simulink model "frbd_64ch_600mhz"  (R2013b)
(part 3 of 148)

  pipeline93 : Subsystem  AncestorBlock=casper_library_delays/pipeline  mask(pipeline){latency=1}
      mask help:
      | An explicitly laid-out delay line to avoid mapping to SRL16s
      | for use in pipelining to help achieve timing closure.
      mask init:
      | pipeline_init(gcb,'latency',latency);
      settings: AttributesFormatString=Latency = %<latency>
      mask Display:
      | port_label('input', 1, 'd');
      | port_label('output', 1, 'q');
      | disp(['Z^-', num2str(latency)]);
  pipeline94 : Subsystem  AncestorBlock=casper_library_delays/pipeline  mask(pipeline){latency=1}
      mask help:
      | An explicitly laid-out delay line to avoid mapping to SRL16s
      | for use in pipelining to help achieve timing closure.
      mask init:
      | pipeline_init(gcb,'latency',latency);
      settings: AttributesFormatString=Latency = %<latency>
      mask Display:
      | port_label('input', 1, 'd');
      | port_label('output', 1, 'q');
      | disp(['Z^-', num2str(latency)]);
  pipeline95 : Subsystem  AncestorBlock=casper_library_delays/pipeline  mask(pipeline){latency=1}
      mask help:
      | An explicitly laid-out delay line to avoid mapping to SRL16s
      | for use in pipelining to help achieve timing closure.
      mask init:
      | pipeline_init(gcb,'latency',latency);
      settings: AttributesFormatString=Latency = %<latency>
      mask Display:
      | port_label('input', 1, 'd');
      | port_label('output', 1, 'q');
      | disp(['Z^-', num2str(latency)]);
  pipeline96 : Subsystem  AncestorBlock=casper_library_delays/pipeline  mask(pipeline){latency=1}
      mask help:
      | An explicitly laid-out delay line to avoid mapping to SRL16s
      | for use in pipelining to help achieve timing closure.
      mask init:
      | pipeline_init(gcb,'latency',latency);
      settings: AttributesFormatString=Latency = %<latency>
      mask Display:
      | port_label('input', 1, 'd');
      | port_label('output', 1, 'q');
      | disp(['Z^-', num2str(latency)]);
  pipeline97 : Subsystem  AncestorBlock=casper_library_delays/pipeline  mask(pipeline){latency=1}
      mask help:
      | An explicitly laid-out delay line to avoid mapping to SRL16s
      | for use in pipelining to help achieve timing closure.
      mask init:
      | pipeline_init(gcb,'latency',latency);
      settings: AttributesFormatString=Latency = %<latency>
      mask Display:
      | port_label('input', 1, 'd');
      | port_label('output', 1, 'q');
      | disp(['Z^-', num2str(latency)]);
  pipeline98 : Subsystem  AncestorBlock=casper_library_delays/pipeline  mask(pipeline){latency=1}
      mask help:
      | An explicitly laid-out delay line to avoid mapping to SRL16s
      | for use in pipelining to help achieve timing closure.
      mask init:
      | pipeline_init(gcb,'latency',latency);
      settings: AttributesFormatString=Latency = %<latency>
      mask Display:
      | port_label('input', 1, 'd');
      | port_label('output', 1, 'q');
      | disp(['Z^-', num2str(latency)]);
  pipeline99 : Subsystem  AncestorBlock=casper_library_delays/pipeline  mask(pipeline){latency=1}
      mask help:
      | An explicitly laid-out delay line to avoid mapping to SRL16s
      | for use in pipelining to help achieve timing closure.
      mask init:
      | pipeline_init(gcb,'latency',latency);
      settings: AttributesFormatString=Latency = %<latency>
      mask Display:
      | port_label('input', 1, 'd');
      | port_label('output', 1, 'q');
      | disp(['Z^-', num2str(latency)]);
  power{1..4} (4 alike) : casper_library_misc/power  BitWidth=18  add_latency=2  mult_latency=3
  ring : Subsystem
  simple_bram_vacc : Subsystem  AncestorBlock=casper_library_accumulators/simple_bram_vacc  mask(simple_bram_vacc){vec_len=16, arith_type=Unsigned, n_bits=26, bin_pt=7}
      mask prompts: vec_len "Vector length:"; arith_type "Output type:"; n_bits "Bit width (output):"; bin_pt "Binary point (output):"
      mask help: This simple vector accumulator is based on a shift register. It outputs its previous accumulated vector after a new_acc pulse is received.
      mask init:
      | simple_bram_vacc_init(gcb, ...
      |     'vec_len', vec_len, ...
      |     'arith_type', arith_type, ...
      |     'n_bits', n_bits, ...
      |     'bin_pt', bin_pt);
      mask TypeOptions arith_type: Signed | Unsigned
  simple_bram_vacc1 : Subsystem  AncestorBlock=casper_library_accumulators/simple_bram_vacc  mask(simple_bram_vacc){vec_len=16, arith_type=Unsigned, n_bits=26, bin_pt=7}
      mask prompts: vec_len "Vector length:"; arith_type "Output type:"; n_bits "Bit width (output):"; bin_pt "Binary point (output):"
      mask help: This simple vector accumulator is based on a shift register. It outputs its previous accumulated vector after a new_acc pulse is received.
      mask init:
      | simple_bram_vacc_init(gcb, ...
      |     'vec_len', vec_len, ...
      |     'arith_type', arith_type, ...
      |     'n_bits', n_bits, ...
      |     'bin_pt', bin_pt);
      mask TypeOptions arith_type: Signed | Unsigned
  simple_bram_vacc10 : Subsystem  AncestorBlock=casper_library_accumulators/simple_bram_vacc  mask(simple_bram_vacc){vec_len=16, arith_type=Unsigned, n_bits=26, bin_pt=7}
      mask prompts: vec_len "Vector length:"; arith_type "Output type:"; n_bits "Bit width (output):"; bin_pt "Binary point (output):"
      mask help: This simple vector accumulator is based on a shift register. It outputs its previous accumulated vector after a new_acc pulse is received.
      mask init:
      | simple_bram_vacc_init(gcb, ...
      |     'vec_len', vec_len, ...
      |     'arith_type', arith_type, ...
      |     'n_bits', n_bits, ...
      |     'bin_pt', bin_pt);
      mask TypeOptions arith_type: Signed | Unsigned
  simple_bram_vacc11 : Subsystem  AncestorBlock=casper_library_accumulators/simple_bram_vacc  mask(simple_bram_vacc){vec_len=16, arith_type=Unsigned, n_bits=26, bin_pt=7}
      mask prompts: vec_len "Vector length:"; arith_type "Output type:"; n_bits "Bit width (output):"; bin_pt "Binary point (output):"
      mask help: This simple vector accumulator is based on a shift register. It outputs its previous accumulated vector after a new_acc pulse is received.
      mask init:
      | simple_bram_vacc_init(gcb, ...
      |     'vec_len', vec_len, ...
      |     'arith_type', arith_type, ...
      |     'n_bits', n_bits, ...
      |     'bin_pt', bin_pt);
      mask TypeOptions arith_type: Signed | Unsigned
  simple_bram_vacc12 : Subsystem  AncestorBlock=casper_library_accumulators/simple_bram_vacc  mask(simple_bram_vacc){vec_len=16, arith_type=Unsigned, n_bits=26, bin_pt=7}
      mask prompts: vec_len "Vector length:"; arith_type "Output type:"; n_bits "Bit width (output):"; bin_pt "Binary point (output):"
      mask help: This simple vector accumulator is based on a shift register. It outputs its previous accumulated vector after a new_acc pulse is received.
      mask init:
      | simple_bram_vacc_init(gcb, ...
      |     'vec_len', vec_len, ...
      |     'arith_type', arith_type, ...
      |     'n_bits', n_bits, ...
      |     'bin_pt', bin_pt);
      mask TypeOptions arith_type: Signed | Unsigned
  simple_bram_vacc13 : Subsystem  AncestorBlock=casper_library_accumulators/simple_bram_vacc  mask(simple_bram_vacc){vec_len=16, arith_type=Unsigned, n_bits=26, bin_pt=7}
      mask prompts: vec_len "Vector length:"; arith_type "Output type:"; n_bits "Bit width (output):"; bin_pt "Binary point (output):"
      mask help: This simple vector accumulator is based on a shift register. It outputs its previous accumulated vector after a new_acc pulse is received.
      mask init:
      | simple_bram_vacc_init(gcb, ...
      |     'vec_len', vec_len, ...
      |     'arith_type', arith_type, ...
      |     'n_bits', n_bits, ...
      |     'bin_pt', bin_pt);
      mask TypeOptions arith_type: Signed | Unsigned
  simple_bram_vacc14 : Subsystem  AncestorBlock=casper_library_accumulators/simple_bram_vacc  mask(simple_bram_vacc){vec_len=16, arith_type=Unsigned, n_bits=26, bin_pt=7}
      mask prompts: vec_len "Vector length:"; arith_type "Output type:"; n_bits "Bit width (output):"; bin_pt "Binary point (output):"
      mask help: This simple vector accumulator is based on a shift register. It outputs its previous accumulated vector after a new_acc pulse is received.
      mask init:
      | simple_bram_vacc_init(gcb, ...
      |     'vec_len', vec_len, ...
      |     'arith_type', arith_type, ...
      |     'n_bits', n_bits, ...
      |     'bin_pt', bin_pt);
      mask TypeOptions arith_type: Signed | Unsigned
  simple_bram_vacc15 : Subsystem  AncestorBlock=casper_library_accumulators/simple_bram_vacc  mask(simple_bram_vacc){vec_len=16, arith_type=Unsigned, n_bits=26, bin_pt=7}
      mask prompts: vec_len "Vector length:"; arith_type "Output type:"; n_bits "Bit width (output):"; bin_pt "Binary point (output):"
      mask help: This simple vector accumulator is based on a shift register. It outputs its previous accumulated vector after a new_acc pulse is received.
      mask init:
      | simple_bram_vacc_init(gcb, ...
      |     'vec_len', vec_len, ...
      |     'arith_type', arith_type, ...
      |     'n_bits', n_bits, ...
      |     'bin_pt', bin_pt);
      mask TypeOptions arith_type: Signed | Unsigned
  simple_bram_vacc16 : Subsystem  AncestorBlock=casper_library_accumulators/simple_bram_vacc  mask(simple_bram_vacc){vec_len=16, arith_type=Unsigned, n_bits=26, bin_pt=7}
      mask prompts: vec_len "Vector length:"; arith_type "Output type:"; n_bits "Bit width (output):"; bin_pt "Binary point (output):"
      mask help: This simple vector accumulator is based on a shift register. It outputs its previous accumulated vector after a new_acc pulse is received.
      mask init:
      | simple_bram_vacc_init(gcb, ...
      |     'vec_len', vec_len, ...
      |     'arith_type', arith_type, ...
      |     'n_bits', n_bits, ...
      |     'bin_pt', bin_pt);
      mask TypeOptions arith_type: Signed | Unsigned
  simple_bram_vacc17 : Subsystem  AncestorBlock=casper_library_accumulators/simple_bram_vacc  mask(simple_bram_vacc){vec_len=16, arith_type=Unsigned, n_bits=26, bin_pt=7}
      mask prompts: vec_len "Vector length:"; arith_type "Output type:"; n_bits "Bit width (output):"; bin_pt "Binary point (output):"
      mask help: This simple vector accumulator is based on a shift register. It outputs its previous accumulated vector after a new_acc pulse is received.
      mask init:
      | simple_bram_vacc_init(gcb, ...
      |     'vec_len', vec_len, ...
      |     'arith_type', arith_type, ...
      |     'n_bits', n_bits, ...
      |     'bin_pt', bin_pt);
      mask TypeOptions arith_type: Signed | Unsigned
  simple_bram_vacc18 : Subsystem  AncestorBlock=casper_library_accumulators/simple_bram_vacc  mask(simple_bram_vacc){vec_len=16, arith_type=Unsigned, n_bits=26, bin_pt=7}
      mask prompts: vec_len "Vector length:"; arith_type "Output type:"; n_bits "Bit width (output):"; bin_pt "Binary point (output):"
      mask help: This simple vector accumulator is based on a shift register. It outputs its previous accumulated vector after a new_acc pulse is received.
      mask init:
      | simple_bram_vacc_init(gcb, ...
      |     'vec_len', vec_len, ...
      |     'arith_type', arith_type, ...
      |     'n_bits', n_bits, ...
      |     'bin_pt', bin_pt);
      mask TypeOptions arith_type: Signed | Unsigned
  simple_bram_vacc19 : Subsystem  AncestorBlock=casper_library_accumulators/simple_bram_vacc  mask(simple_bram_vacc){vec_len=16, arith_type=Unsigned, n_bits=26, bin_pt=7}
      mask prompts: vec_len "Vector length:"; arith_type "Output type:"; n_bits "Bit width (output):"; bin_pt "Binary point (output):"
      mask help: This simple vector accumulator is based on a shift register. It outputs its previous accumulated vector after a new_acc pulse is received.
      mask init:
      | simple_bram_vacc_init(gcb, ...
      |     'vec_len', vec_len, ...
      |     'arith_type', arith_type, ...
      |     'n_bits', n_bits, ...
      |     'bin_pt', bin_pt);
      mask TypeOptions arith_type: Signed | Unsigned
  simple_bram_vacc2 : Subsystem  AncestorBlock=casper_library_accumulators/simple_bram_vacc  mask(simple_bram_vacc){vec_len=16, arith_type=Unsigned, n_bits=26, bin_pt=7}
      mask prompts: vec_len "Vector length:"; arith_type "Output type:"; n_bits "Bit width (output):"; bin_pt "Binary point (output):"
      mask help: This simple vector accumulator is based on a shift register. It outputs its previous accumulated vector after a new_acc pulse is received.
      mask init:
      | simple_bram_vacc_init(gcb, ...
      |     'vec_len', vec_len, ...
      |     'arith_type', arith_type, ...
      |     'n_bits', n_bits, ...
      |     'bin_pt', bin_pt);
      mask TypeOptions arith_type: Signed | Unsigned
  simple_bram_vacc20 : Subsystem  AncestorBlock=casper_library_accumulators/simple_bram_vacc  mask(simple_bram_vacc){vec_len=16, arith_type=Unsigned, n_bits=26, bin_pt=7}
      mask prompts: vec_len "Vector length:"; arith_type "Output type:"; n_bits "Bit width (output):"; bin_pt "Binary point (output):"
      mask help: This simple vector accumulator is based on a shift register. It outputs its previous accumulated vector after a new_acc pulse is received.
      mask init:
      | simple_bram_vacc_init(gcb, ...
      |     'vec_len', vec_len, ...
      |     'arith_type', arith_type, ...
      |     'n_bits', n_bits, ...
      |     'bin_pt', bin_pt);
      mask TypeOptions arith_type: Signed | Unsigned
  simple_bram_vacc21 : Subsystem  AncestorBlock=casper_library_accumulators/simple_bram_vacc  mask(simple_bram_vacc){vec_len=16, arith_type=Unsigned, n_bits=26, bin_pt=7}
      mask prompts: vec_len "Vector length:"; arith_type "Output type:"; n_bits "Bit width (output):"; bin_pt "Binary point (output):"
      mask help: This simple vector accumulator is based on a shift register. It outputs its previous accumulated vector after a new_acc pulse is received.
      mask init:
      | simple_bram_vacc_init(gcb, ...
      |     'vec_len', vec_len, ...
      |     'arith_type', arith_type, ...
      |     'n_bits', n_bits, ...
      |     'bin_pt', bin_pt);
      mask TypeOptions arith_type: Signed | Unsigned
  simple_bram_vacc22 : Subsystem  AncestorBlock=casper_library_accumulators/simple_bram_vacc  mask(simple_bram_vacc){vec_len=16, arith_type=Unsigned, n_bits=26, bin_pt=7}
      mask prompts: vec_len "Vector length:"; arith_type "Output type:"; n_bits "Bit width (output):"; bin_pt "Binary point (output):"
      mask help: This simple vector accumulator is based on a shift register. It outputs its previous accumulated vector after a new_acc pulse is received.
      mask init:
      | simple_bram_vacc_init(gcb, ...
      |     'vec_len', vec_len, ...
      |     'arith_type', arith_type, ...
      |     'n_bits', n_bits, ...
      |     'bin_pt', bin_pt);
      mask TypeOptions arith_type: Signed | Unsigned
  simple_bram_vacc23 : Subsystem  AncestorBlock=casper_library_accumulators/simple_bram_vacc  mask(simple_bram_vacc){vec_len=16, arith_type=Unsigned, n_bits=26, bin_pt=7}
      mask prompts: vec_len "Vector length:"; arith_type "Output type:"; n_bits "Bit width (output):"; bin_pt "Binary point (output):"
      mask help: This simple vector accumulator is based on a shift register. It outputs its previous accumulated vector after a new_acc pulse is received.
      mask init:
      | simple_bram_vacc_init(gcb, ...
      |     'vec_len', vec_len, ...
      |     'arith_type', arith_type, ...
      |     'n_bits', n_bits, ...
      |     'bin_pt', bin_pt);
      mask TypeOptions arith_type: Signed | Unsigned
  simple_bram_vacc24 : Subsystem  AncestorBlock=casper_library_accumulators/simple_bram_vacc  mask(simple_bram_vacc){vec_len=16, arith_type=Unsigned, n_bits=26, bin_pt=7}
      mask prompts: vec_len "Vector length:"; arith_type "Output type:"; n_bits "Bit width (output):"; bin_pt "Binary point (output):"
      mask help: This simple vector accumulator is based on a shift register. It outputs its previous accumulated vector after a new_acc pulse is received.
      mask init:
      | simple_bram_vacc_init(gcb, ...
      |     'vec_len', vec_len, ...
      |     'arith_type', arith_type, ...
      |     'n_bits', n_bits, ...
      |     'bin_pt', bin_pt);
      mask TypeOptions arith_type: Signed | Unsigned
  simple_bram_vacc25 : Subsystem  AncestorBlock=casper_library_accumulators/simple_bram_vacc  mask(simple_bram_vacc){vec_len=16, arith_type=Unsigned, n_bits=26, bin_pt=7}
      mask prompts: vec_len "Vector length:"; arith_type "Output type:"; n_bits "Bit width (output):"; bin_pt "Binary point (output):"
      mask help: This simple vector accumulator is based on a shift register. It outputs its previous accumulated vector after a new_acc pulse is received.
      mask init:
      | simple_bram_vacc_init(gcb, ...
      |     'vec_len', vec_len, ...
      |     'arith_type', arith_type, ...
      |     'n_bits', n_bits, ...
      |     'bin_pt', bin_pt);
      mask TypeOptions arith_type: Signed | Unsigned
  simple_bram_vacc26 : Subsystem  AncestorBlock=casper_library_accumulators/simple_bram_vacc  mask(simple_bram_vacc){vec_len=16, arith_type=Unsigned, n_bits=26, bin_pt=7}
      mask prompts: vec_len "Vector length:"; arith_type "Output type:"; n_bits "Bit width (output):"; bin_pt "Binary point (output):"
      mask help: This simple vector accumulator is based on a shift register. It outputs its previous accumulated vector after a new_acc pulse is received.
      mask init:
      | simple_bram_vacc_init(gcb, ...
      |     'vec_len', vec_len, ...
      |     'arith_type', arith_type, ...
      |     'n_bits', n_bits, ...
      |     'bin_pt', bin_pt);
      mask TypeOptions arith_type: Signed | Unsigned
  simple_bram_vacc27 : Subsystem  AncestorBlock=casper_library_accumulators/simple_bram_vacc  mask(simple_bram_vacc){vec_len=16, arith_type=Unsigned, n_bits=26, bin_pt=7}
      mask prompts: vec_len "Vector length:"; arith_type "Output type:"; n_bits "Bit width (output):"; bin_pt "Binary point (output):"
      mask help: This simple vector accumulator is based on a shift register. It outputs its previous accumulated vector after a new_acc pulse is received.
      mask init:
      | simple_bram_vacc_init(gcb, ...
      |     'vec_len', vec_len, ...
      |     'arith_type', arith_type, ...
      |     'n_bits', n_bits, ...
      |     'bin_pt', bin_pt);
      mask TypeOptions arith_type: Signed | Unsigned
  simple_bram_vacc28 : Subsystem  AncestorBlock=casper_library_accumulators/simple_bram_vacc  mask(simple_bram_vacc){vec_len=16, arith_type=Unsigned, n_bits=26, bin_pt=7}
      mask prompts: vec_len "Vector length:"; arith_type "Output type:"; n_bits "Bit width (output):"; bin_pt "Binary point (output):"
      mask help: This simple vector accumulator is based on a shift register. It outputs its previous accumulated vector after a new_acc pulse is received.
      mask init:
      | simple_bram_vacc_init(gcb, ...
      |     'vec_len', vec_len, ...
      |     'arith_type', arith_type, ...
      |     'n_bits', n_bits, ...
      |     'bin_pt', bin_pt);
      mask TypeOptions arith_type: Signed | Unsigned
  simple_bram_vacc29 : Subsystem  AncestorBlock=casper_library_accumulators/simple_bram_vacc  mask(simple_bram_vacc){vec_len=16, arith_type=Unsigned, n_bits=26, bin_pt=7}
      mask prompts: vec_len "Vector length:"; arith_type "Output type:"; n_bits "Bit width (output):"; bin_pt "Binary point (output):"
      mask help: This simple vector accumulator is based on a shift register. It outputs its previous accumulated vector after a new_acc pulse is received.
      mask init:
      | simple_bram_vacc_init(gcb, ...
      |     'vec_len', vec_len, ...
      |     'arith_type', arith_type, ...
      |     'n_bits', n_bits, ...
      |     'bin_pt', bin_pt);
      mask TypeOptions arith_type: Signed | Unsigned
  simple_bram_vacc3 : Subsystem  AncestorBlock=casper_library_accumulators/simple_bram_vacc  mask(simple_bram_vacc){vec_len=16, arith_type=Unsigned, n_bits=26, bin_pt=7}
      mask prompts: vec_len "Vector length:"; arith_type "Output type:"; n_bits "Bit width (output):"; bin_pt "Binary point (output):"
      mask help: This simple vector accumulator is based on a shift register. It outputs its previous accumulated vector after a new_acc pulse is received.
      mask init:
      | simple_bram_vacc_init(gcb, ...
      |     'vec_len', vec_len, ...
      |     'arith_type', arith_type, ...
      |     'n_bits', n_bits, ...
      |     'bin_pt', bin_pt);
      mask TypeOptions arith_type: Signed | Unsigned
  simple_bram_vacc30 : Subsystem  AncestorBlock=casper_library_accumulators/simple_bram_vacc  mask(simple_bram_vacc){vec_len=16, arith_type=Unsigned, n_bits=26, bin_pt=7}
      mask prompts: vec_len "Vector length:"; arith_type "Output type:"; n_bits "Bit width (output):"; bin_pt "Binary point (output):"
      mask help: This simple vector accumulator is based on a shift register. It outputs its previous accumulated vector after a new_acc pulse is received.
      mask init:
      | simple_bram_vacc_init(gcb, ...
      |     'vec_len', vec_len, ...
      |     'arith_type', arith_type, ...
      |     'n_bits', n_bits, ...
      |     'bin_pt', bin_pt);
      mask TypeOptions arith_type: Signed | Unsigned
  simple_bram_vacc31 : Subsystem  AncestorBlock=casper_library_accumulators/simple_bram_vacc  mask(simple_bram_vacc){vec_len=16, arith_type=Unsigned, n_bits=26, bin_pt=7}
      mask prompts: vec_len "Vector length:"; arith_type "Output type:"; n_bits "Bit width (output):"; bin_pt "Binary point (output):"
      mask help: This simple vector accumulator is based on a shift register. It outputs its previous accumulated vector after a new_acc pulse is received.
      mask init:
      | simple_bram_vacc_init(gcb, ...
      |     'vec_len', vec_len, ...
      |     'arith_type', arith_type, ...
      |     'n_bits', n_bits, ...
      |     'bin_pt', bin_pt);
      mask TypeOptions arith_type: Signed | Unsigned
  simple_bram_vacc32 : Subsystem  AncestorBlock=casper_library_accumulators/simple_bram_vacc  mask(simple_bram_vacc){vec_len=16, arith_type=Unsigned, n_bits=26, bin_pt=7}
      mask prompts: vec_len "Vector length:"; arith_type "Output type:"; n_bits "Bit width (output):"; bin_pt "Binary point (output):"
      mask help: This simple vector accumulator is based on a shift register. It outputs its previous accumulated vector after a new_acc pulse is received.
      mask init:
      | simple_bram_vacc_init(gcb, ...
      |     'vec_len', vec_len, ...
      |     'arith_type', arith_type, ...
      |     'n_bits', n_bits, ...
      |     'bin_pt', bin_pt);
      mask TypeOptions arith_type: Signed | Unsigned
  simple_bram_vacc33 : Subsystem  AncestorBlock=casper_library_accumulators/simple_bram_vacc  mask(simple_bram_vacc){vec_len=16, arith_type=Unsigned, n_bits=26, bin_pt=7}
      mask prompts: vec_len "Vector length:"; arith_type "Output type:"; n_bits "Bit width (output):"; bin_pt "Binary point (output):"
      mask help: This simple vector accumulator is based on a shift register. It outputs its previous accumulated vector after a new_acc pulse is received.
      mask init:
      | simple_bram_vacc_init(gcb, ...
      |     'vec_len', vec_len, ...
      |     'arith_type', arith_type, ...
      |     'n_bits', n_bits, ...
      |     'bin_pt', bin_pt);
      mask TypeOptions arith_type: Signed | Unsigned
  simple_bram_vacc34 : Subsystem  AncestorBlock=casper_library_accumulators/simple_bram_vacc  mask(simple_bram_vacc){vec_len=16, arith_type=Unsigned, n_bits=26, bin_pt=7}
      mask prompts: vec_len "Vector length:"; arith_type "Output type:"; n_bits "Bit width (output):"; bin_pt "Binary point (output):"
      mask help: This simple vector accumulator is based on a shift register. It outputs its previous accumulated vector after a new_acc pulse is received.
      mask init:
      | simple_bram_vacc_init(gcb, ...
      |     'vec_len', vec_len, ...
      |     'arith_type', arith_type, ...
      |     'n_bits', n_bits, ...
      |     'bin_pt', bin_pt);
      mask TypeOptions arith_type: Signed | Unsigned
  simple_bram_vacc35 : Subsystem  AncestorBlock=casper_library_accumulators/simple_bram_vacc  mask(simple_bram_vacc){vec_len=16, arith_type=Unsigned, n_bits=26, bin_pt=7}
      mask prompts: vec_len "Vector length:"; arith_type "Output type:"; n_bits "Bit width (output):"; bin_pt "Binary point (output):"
      mask help: This simple vector accumulator is based on a shift register. It outputs its previous accumulated vector after a new_acc pulse is received.
      mask init:
      | simple_bram_vacc_init(gcb, ...
      |     'vec_len', vec_len, ...
      |     'arith_type', arith_type, ...
      |     'n_bits', n_bits, ...
      |     'bin_pt', bin_pt);
      mask TypeOptions arith_type: Signed | Unsigned
  simple_bram_vacc36 : Subsystem  AncestorBlock=casper_library_accumulators/simple_bram_vacc  mask(simple_bram_vacc){vec_len=16, arith_type=Unsigned, n_bits=26, bin_pt=7}
      mask prompts: vec_len "Vector length:"; arith_type "Output type:"; n_bits "Bit width (output):"; bin_pt "Binary point (output):"
      mask help: This simple vector accumulator is based on a shift register. It outputs its previous accumulated vector after a new_acc pulse is received.
      mask init:
      | simple_bram_vacc_init(gcb, ...
      |     'vec_len', vec_len, ...
      |     'arith_type', arith_type, ...
      |     'n_bits', n_bits, ...
      |     'bin_pt', bin_pt);
      mask TypeOptions arith_type: Signed | Unsigned
  simple_bram_vacc37 : Subsystem  AncestorBlock=casper_library_accumulators/simple_bram_vacc  mask(simple_bram_vacc){vec_len=16, arith_type=Unsigned, n_bits=26, bin_pt=7}
      mask prompts: vec_len "Vector length:"; arith_type "Output type:"; n_bits "Bit width (output):"; bin_pt "Binary point (output):"
      mask help: This simple vector accumulator is based on a shift register. It outputs its previous accumulated vector after a new_acc pulse is received.
      mask init:
      | simple_bram_vacc_init(gcb, ...
      |     'vec_len', vec_len, ...
      |     'arith_type', arith_type, ...
      |     'n_bits', n_bits, ...
      |     'bin_pt', bin_pt);
      mask TypeOptions arith_type: Signed | Unsigned
  simple_bram_vacc38 : Subsystem  AncestorBlock=casper_library_accumulators/simple_bram_vacc  mask(simple_bram_vacc){vec_len=16, arith_type=Unsigned, n_bits=26, bin_pt=7}
      mask prompts: vec_len "Vector length:"; arith_type "Output type:"; n_bits "Bit width (output):"; bin_pt "Binary point (output):"
      mask help: This simple vector accumulator is based on a shift register. It outputs its previous accumulated vector after a new_acc pulse is received.
      mask init:
      | simple_bram_vacc_init(gcb, ...
      |     'vec_len', vec_len, ...
      |     'arith_type', arith_type, ...
      |     'n_bits', n_bits, ...
      |     'bin_pt', bin_pt);
      mask TypeOptions arith_type: Signed | Unsigned
  simple_bram_vacc39 : Subsystem  AncestorBlock=casper_library_accumulators/simple_bram_vacc  mask(simple_bram_vacc){vec_len=16, arith_type=Unsigned, n_bits=26, bin_pt=7}
      mask prompts: vec_len "Vector length:"; arith_type "Output type:"; n_bits "Bit width (output):"; bin_pt "Binary point (output):"
      mask help: This simple vector accumulator is based on a shift register. It outputs its previous accumulated vector after a new_acc pulse is received.
      mask init:
      | simple_bram_vacc_init(gcb, ...
      |     'vec_len', vec_len, ...
      |     'arith_type', arith_type, ...
      |     'n_bits', n_bits, ...
      |     'bin_pt', bin_pt);
      mask TypeOptions arith_type: Signed | Unsigned
  simple_bram_vacc4 : Subsystem  AncestorBlock=casper_library_accumulators/simple_bram_vacc  mask(simple_bram_vacc){vec_len=16, arith_type=Unsigned, n_bits=26, bin_pt=7}
      mask prompts: vec_len "Vector length:"; arith_type "Output type:"; n_bits "Bit width (output):"; bin_pt "Binary point (output):"
      mask help: This simple vector accumulator is based on a shift register. It outputs its previous accumulated vector after a new_acc pulse is received.
      mask init:
      | simple_bram_vacc_init(gcb, ...
      |     'vec_len', vec_len, ...
      |     'arith_type', arith_type, ...
      |     'n_bits', n_bits, ...
      |     'bin_pt', bin_pt);
      mask TypeOptions arith_type: Signed | Unsigned
  simple_bram_vacc40 : Subsystem  AncestorBlock=casper_library_accumulators/simple_bram_vacc  mask(simple_bram_vacc){vec_len=16, arith_type=Unsigned, n_bits=26, bin_pt=7}
      mask prompts: vec_len "Vector length:"; arith_type "Output type:"; n_bits "Bit width (output):"; bin_pt "Binary point (output):"
      mask help: This simple vector accumulator is based on a shift register. It outputs its previous accumulated vector after a new_acc pulse is received.
      mask init:
      | simple_bram_vacc_init(gcb, ...
      |     'vec_len', vec_len, ...
      |     'arith_type', arith_type, ...
      |     'n_bits', n_bits, ...
      |     'bin_pt', bin_pt);
      mask TypeOptions arith_type: Signed | Unsigned
  simple_bram_vacc41 : Subsystem  AncestorBlock=casper_library_accumulators/simple_bram_vacc  mask(simple_bram_vacc){vec_len=16, arith_type=Unsigned, n_bits=26, bin_pt=7}
      mask prompts: vec_len "Vector length:"; arith_type "Output type:"; n_bits "Bit width (output):"; bin_pt "Binary point (output):"
      mask help: This simple vector accumulator is based on a shift register. It outputs its previous accumulated vector after a new_acc pulse is received.
      mask init:
      | simple_bram_vacc_init(gcb, ...
      |     'vec_len', vec_len, ...
      |     'arith_type', arith_type, ...
      |     'n_bits', n_bits, ...
      |     'bin_pt', bin_pt);
      mask TypeOptions arith_type: Signed | Unsigned
  simple_bram_vacc42 : Subsystem  AncestorBlock=casper_library_accumulators/simple_bram_vacc  mask(simple_bram_vacc){vec_len=16, arith_type=Unsigned, n_bits=26, bin_pt=7}
      mask prompts: vec_len "Vector length:"; arith_type "Output type:"; n_bits "Bit width (output):"; bin_pt "Binary point (output):"
      mask help: This simple vector accumulator is based on a shift register. It outputs its previous accumulated vector after a new_acc pulse is received.
      mask init:
      | simple_bram_vacc_init(gcb, ...
      |     'vec_len', vec_len, ...
      |     'arith_type', arith_type, ...
      |     'n_bits', n_bits, ...
      |     'bin_pt', bin_pt);
      mask TypeOptions arith_type: Signed | Unsigned
  simple_bram_vacc43 : Subsystem  AncestorBlock=casper_library_accumulators/simple_bram_vacc  mask(simple_bram_vacc){vec_len=16, arith_type=Unsigned, n_bits=64, bin_pt=35}
      mask prompts: vec_len "Vector length:"; arith_type "Output type:"; n_bits "Bit width (output):"; bin_pt "Binary point (output):"
      mask help: This simple vector accumulator is based on a shift register. It outputs its previous accumulated vector after a new_acc pulse is received.
      mask init:
      | simple_bram_vacc_init(gcb, ...
      |     'vec_len', vec_len, ...
      |     'arith_type', arith_type, ...
      |     'n_bits', n_bits, ...
      |     'bin_pt', bin_pt);
      mask TypeOptions arith_type: Signed | Unsigned
  simple_bram_vacc44 : Subsystem  AncestorBlock=casper_library_accumulators/simple_bram_vacc  mask(simple_bram_vacc){vec_len=16, arith_type=Unsigned, n_bits=64, bin_pt=35}
      mask prompts: vec_len "Vector length:"; arith_type "Output type:"; n_bits "Bit width (output):"; bin_pt "Binary point (output):"
      mask help: This simple vector accumulator is based on a shift register. It outputs its previous accumulated vector after a new_acc pulse is received.
      mask init:
      | simple_bram_vacc_init(gcb, ...
      |     'vec_len', vec_len, ...
      |     'arith_type', arith_type, ...
      |     'n_bits', n_bits, ...
      |     'bin_pt', bin_pt);
      mask TypeOptions arith_type: Signed | Unsigned
  simple_bram_vacc45 : Subsystem  AncestorBlock=casper_library_accumulators/simple_bram_vacc  mask(simple_bram_vacc){vec_len=16, arith_type=Unsigned, n_bits=64, bin_pt=35}
      mask prompts: vec_len "Vector length:"; arith_type "Output type:"; n_bits "Bit width (output):"; bin_pt "Binary point (output):"
      mask help: This simple vector accumulator is based on a shift register. It outputs its previous accumulated vector after a new_acc pulse is received.
      mask init:
      | simple_bram_vacc_init(gcb, ...
      |     'vec_len', vec_len, ...
      |     'arith_type', arith_type, ...
      |     'n_bits', n_bits, ...
      |     'bin_pt', bin_pt);
      mask TypeOptions arith_type: Signed | Unsigned
  simple_bram_vacc46 : Subsystem  AncestorBlock=casper_library_accumulators/simple_bram_vacc  mask(simple_bram_vacc){vec_len=16, arith_type=Unsigned, n_bits=64, bin_pt=35}
      mask prompts: vec_len "Vector length:"; arith_type "Output type:"; n_bits "Bit width (output):"; bin_pt "Binary point (output):"
      mask help: This simple vector accumulator is based on a shift register. It outputs its previous accumulated vector after a new_acc pulse is received.
      mask init:
      | simple_bram_vacc_init(gcb, ...
      |     'vec_len', vec_len, ...
      |     'arith_type', arith_type, ...
      |     'n_bits', n_bits, ...
      |     'bin_pt', bin_pt);
      mask TypeOptions arith_type: Signed | Unsigned
  simple_bram_vacc47 : Subsystem  AncestorBlock=casper_library_accumulators/simple_bram_vacc  mask(simple_bram_vacc){vec_len=16, arith_type=Unsigned, n_bits=26, bin_pt=7}
      mask prompts: vec_len "Vector length:"; arith_type "Output type:"; n_bits "Bit width (output):"; bin_pt "Binary point (output):"
      mask help: This simple vector accumulator is based on a shift register. It outputs its previous accumulated vector after a new_acc pulse is received.
      mask init:
      | simple_bram_vacc_init(gcb, ...
      |     'vec_len', vec_len, ...
      |     'arith_type', arith_type, ...
      |     'n_bits', n_bits, ...
      |     'bin_pt', bin_pt);
      mask TypeOptions arith_type: Signed | Unsigned
  simple_bram_vacc48 : Subsystem  AncestorBlock=casper_library_accumulators/simple_bram_vacc  mask(simple_bram_vacc){vec_len=16, arith_type=Unsigned, n_bits=26, bin_pt=7}
      mask prompts: vec_len "Vector length:"; arith_type "Output type:"; n_bits "Bit width (output):"; bin_pt "Binary point (output):"
      mask help: This simple vector accumulator is based on a shift register. It outputs its previous accumulated vector after a new_acc pulse is received.
      mask init:
      | simple_bram_vacc_init(gcb, ...
      |     'vec_len', vec_len, ...
      |     'arith_type', arith_type, ...
      |     'n_bits', n_bits, ...
      |     'bin_pt', bin_pt);
      mask TypeOptions arith_type: Signed | Unsigned
  simple_bram_vacc49 : Subsystem  AncestorBlock=casper_library_accumulators/simple_bram_vacc  mask(simple_bram_vacc){vec_len=16, arith_type=Unsigned, n_bits=26, bin_pt=7}
      mask prompts: vec_len "Vector length:"; arith_type "Output type:"; n_bits "Bit width (output):"; bin_pt "Binary point (output):"
      mask help: This simple vector accumulator is based on a shift register. It outputs its previous accumulated vector after a new_acc pulse is received.
      mask init:
      | simple_bram_vacc_init(gcb, ...
      |     'vec_len', vec_len, ...
      |     'arith_type', arith_type, ...
      |     'n_bits', n_bits, ...
      |     'bin_pt', bin_pt);
      mask TypeOptions arith_type: Signed | Unsigned
  simple_bram_vacc5 : Subsystem  AncestorBlock=casper_library_accumulators/simple_bram_vacc  mask(simple_bram_vacc){vec_len=16, arith_type=Unsigned, n_bits=26, bin_pt=7}
      mask prompts: vec_len "Vector length:"; arith_type "Output type:"; n_bits "Bit width (output):"; bin_pt "Binary point (output):"
      mask help: This simple vector accumulator is based on a shift register. It outputs its previous accumulated vector after a new_acc pulse is received.
      mask init:
      | simple_bram_vacc_init(gcb, ...
      |     'vec_len', vec_len, ...
      |     'arith_type', arith_type, ...
      |     'n_bits', n_bits, ...
      |     'bin_pt', bin_pt);
      mask TypeOptions arith_type: Signed | Unsigned
  simple_bram_vacc50 : Subsystem  AncestorBlock=casper_library_accumulators/simple_bram_vacc  mask(simple_bram_vacc){vec_len=16, arith_type=Unsigned, n_bits=26, bin_pt=7}
      mask prompts: vec_len "Vector length:"; arith_type "Output type:"; n_bits "Bit width (output):"; bin_pt "Binary point (output):"
      mask help: This simple vector accumulator is based on a shift register. It outputs its previous accumulated vector after a new_acc pulse is received.
      mask init:
      | simple_bram_vacc_init(gcb, ...
      |     'vec_len', vec_len, ...
      |     'arith_type', arith_type, ...
      |     'n_bits', n_bits, ...
      |     'bin_pt', bin_pt);
      mask TypeOptions arith_type: Signed | Unsigned
  simple_bram_vacc6 : Subsystem  AncestorBlock=casper_library_accumulators/simple_bram_vacc  mask(simple_bram_vacc){vec_len=16, arith_type=Unsigned, n_bits=26, bin_pt=7}
      mask prompts: vec_len "Vector length:"; arith_type "Output type:"; n_bits "Bit width (output):"; bin_pt "Binary point (output):"
      mask help: This simple vector accumulator is based on a shift register. It outputs its previous accumulated vector after a new_acc pulse is received.
      mask init:
      | simple_bram_vacc_init(gcb, ...
      |     'vec_len', vec_len, ...
      |     'arith_type', arith_type, ...
      |     'n_bits', n_bits, ...
      |     'bin_pt', bin_pt);
      mask TypeOptions arith_type: Signed | Unsigned
  simple_bram_vacc7 : Subsystem  AncestorBlock=casper_library_accumulators/simple_bram_vacc  mask(simple_bram_vacc){vec_len=16, arith_type=Unsigned, n_bits=26, bin_pt=7}
      mask prompts: vec_len "Vector length:"; arith_type "Output type:"; n_bits "Bit width (output):"; bin_pt "Binary point (output):"
      mask help: This simple vector accumulator is based on a shift register. It outputs its previous accumulated vector after a new_acc pulse is received.
      mask init:
      | simple_bram_vacc_init(gcb, ...
      |     'vec_len', vec_len, ...
      |     'arith_type', arith_type, ...
      |     'n_bits', n_bits, ...
      |     'bin_pt', bin_pt);
      mask TypeOptions arith_type: Signed | Unsigned
  simple_bram_vacc8 : Subsystem  AncestorBlock=casper_library_accumulators/simple_bram_vacc  mask(simple_bram_vacc){vec_len=16, arith_type=Unsigned, n_bits=26, bin_pt=7}
      mask prompts: vec_len "Vector length:"; arith_type "Output type:"; n_bits "Bit width (output):"; bin_pt "Binary point (output):"
      mask help: This simple vector accumulator is based on a shift register. It outputs its previous accumulated vector after a new_acc pulse is received.
      mask init:
      | simple_bram_vacc_init(gcb, ...
      |     'vec_len', vec_len, ...
      |     'arith_type', arith_type, ...
      |     'n_bits', n_bits, ...
      |     'bin_pt', bin_pt);
      mask TypeOptions arith_type: Signed | Unsigned
  simple_bram_vacc86 : Subsystem  AncestorBlock=casper_library_accumulators/simple_bram_vacc  mask(simple_bram_vacc){vec_len=16, arith_type=Unsigned, n_bits=26, bin_pt=7}
      mask prompts: vec_len "Vector length:"; arith_type "Output type:"; n_bits "Bit width (output):"; bin_pt "Binary point (output):"
      mask help: This simple vector accumulator is based on a shift register. It outputs its previous accumulated vector after a new_acc pulse is received.
      mask init:
      | simple_bram_vacc_init(gcb, ...
      |     'vec_len', vec_len, ...
      |     'arith_type', arith_type, ...
      |     'n_bits', n_bits, ...
      |     'bin_pt', bin_pt);
      mask TypeOptions arith_type: Signed | Unsigned
  simple_bram_vacc9 : Subsystem  AncestorBlock=casper_library_accumulators/simple_bram_vacc  mask(simple_bram_vacc){vec_len=16, arith_type=Unsigned, n_bits=26, bin_pt=7}
      mask prompts: vec_len "Vector length:"; arith_type "Output type:"; n_bits "Bit width (output):"; bin_pt "Binary point (output):"
      mask help: This simple vector accumulator is based on a shift register. It outputs its previous accumulated vector after a new_acc pulse is received.
      mask init:
      | simple_bram_vacc_init(gcb, ...
      |     'vec_len', vec_len, ...
      |     'arith_type', arith_type, ...
      |     'n_bits', n_bits, ...
      |     'bin_pt', bin_pt);
      mask TypeOptions arith_type: Signed | Unsigned
  spec0_0 : Subsystem  Tag=xps:bram  AncestorBlock=xps_library/Shared_BRAM  mask{arith_type=Unsigned, addr_width=10, data_width=32, reg_prim_output=on, reg_core_output=on, optimization=Minimum_Area, data_bin_pt=0, init_vals=[0:2^10-1], sample_rate=1}
      mask prompts: arith_type "Output Data Type"; addr_width "Address width"; data_width "Data Width"; reg_prim_output "Register Primitive Output"; reg_core_output "Register Core Output"; data_bin_pt "Data Binary Point"; init_vals "Initial values (simulation only)"; sample_rate "Sample rate"
      mask init:
      | shared_bram_mask;
      mask TypeOptions arith_type: Unsigned | Signed  (2's comp)
      mask TypeOptions data_width: 8 | 16 | 32 | 64 | 128
      mask TypeOptions optimization: Minimum_Area | Low_Power
  spec0_1 : Subsystem  Tag=xps:bram  AncestorBlock=xps_library/Shared_BRAM  mask{arith_type=Unsigned, addr_width=10, data_width=32, reg_prim_output=on, reg_core_output=on, optimization=Minimum_Area, data_bin_pt=0, init_vals=[0:2^10-1], sample_rate=1}
      mask prompts: arith_type "Output Data Type"; addr_width "Address width"; data_width "Data Width"; reg_prim_output "Register Primitive Output"; reg_core_output "Register Core Output"; data_bin_pt "Data Binary Point"; init_vals "Initial values (simulation only)"; sample_rate "Sample rate"
      mask init:
      | shared_bram_mask;
      mask TypeOptions arith_type: Unsigned | Signed  (2's comp)
      mask TypeOptions data_width: 8 | 16 | 32 | 64 | 128
      mask TypeOptions optimization: Minimum_Area | Low_Power
  spec0_2 : Subsystem  Tag=xps:bram  AncestorBlock=xps_library/Shared_BRAM  mask{arith_type=Unsigned, addr_width=10, data_width=32, reg_prim_output=on, reg_core_output=on, optimization=Minimum_Area, data_bin_pt=0, init_vals=[0:2^10-1], sample_rate=1}
      mask prompts: arith_type "Output Data Type"; addr_width "Address width"; data_width "Data Width"; reg_prim_output "Register Primitive Output"; reg_core_output "Register Core Output"; data_bin_pt "Data Binary Point"; init_vals "Initial values (simulation only)"; sample_rate "Sample rate"
      mask init:
      | shared_bram_mask;
      mask TypeOptions arith_type: Unsigned | Signed  (2's comp)
      mask TypeOptions data_width: 8 | 16 | 32 | 64 | 128
      mask TypeOptions optimization: Minimum_Area | Low_Power
  spec0_3 : Subsystem  Tag=xps:bram  AncestorBlock=xps_library/Shared_BRAM  mask{arith_type=Unsigned, addr_width=10, data_width=32, reg_prim_output=on, reg_core_output=on, optimization=Minimum_Area, data_bin_pt=0, init_vals=[0:2^10-1], sample_rate=1}
      mask prompts: arith_type "Output Data Type"; addr_width "Address width"; data_width "Data Width"; reg_prim_output "Register Primitive Output"; reg_core_output "Register Core Output"; data_bin_pt "Data Binary Point"; init_vals "Initial values (simulation only)"; sample_rate "Sample rate"
      mask init:
      | shared_bram_mask;
      mask TypeOptions arith_type: Unsigned | Signed  (2's comp)
      mask TypeOptions data_width: 8 | 16 | 32 | 64 | 128
      mask TypeOptions optimization: Minimum_Area | Low_Power
  spec1_0 : Subsystem  Tag=xps:bram  AncestorBlock=xps_library/Shared_BRAM  mask{arith_type=Unsigned, addr_width=9, data_width=64, reg_prim_output=on, reg_core_output=on, optimization=Minimum_Area, data_bin_pt=0, init_vals=[0:2^10-1], sample_rate=1}
      mask prompts: arith_type "Output Data Type"; addr_width "Address width"; data_width "Data Width"; reg_prim_output "Register Primitive Output"; reg_core_output "Register Core Output"; data_bin_pt "Data Binary Point"; init_vals "Initial values (simulation only)"; sample_rate "Sample rate"
      mask init:
      | shared_bram_mask;
      mask TypeOptions arith_type: Unsigned | Signed  (2's comp)
      mask TypeOptions data_width: 8 | 16 | 32 | 64 | 128
      mask TypeOptions optimization: Minimum_Area | Low_Power
  spec1_1 : Subsystem  Tag=xps:bram  AncestorBlock=xps_library/Shared_BRAM  mask{arith_type=Unsigned, addr_width=9, data_width=64, reg_prim_output=on, reg_core_output=on, optimization=Minimum_Area, data_bin_pt=0, init_vals=[0:2^10-1], sample_rate=1}
      mask prompts: arith_type "Output Data Type"; addr_width "Address width"; data_width "Data Width"; reg_prim_output "Register Primitive Output"; reg_core_output "Register Core Output"; data_bin_pt "Data Binary Point"; init_vals "Initial values (simulation only)"; sample_rate "Sample rate"
      mask init:
      | shared_bram_mask;
      mask TypeOptions arith_type: Unsigned | Signed  (2's comp)
      mask TypeOptions data_width: 8 | 16 | 32 | 64 | 128
      mask TypeOptions optimization: Minimum_Area | Low_Power
  spec1_2 : Subsystem  Tag=xps:bram  AncestorBlock=xps_library/Shared_BRAM  mask{arith_type=Unsigned, addr_width=9, data_width=64, reg_prim_output=on, reg_core_output=on, optimization=Minimum_Area, data_bin_pt=0, init_vals=[0:2^10-1], sample_rate=1}
      mask prompts: arith_type "Output Data Type"; addr_width "Address width"; data_width "Data Width"; reg_prim_output "Register Primitive Output"; reg_core_output "Register Core Output"; data_bin_pt "Data Binary Point"; init_vals "Initial values (simulation only)"; sample_rate "Sample rate"
      mask init:
      | shared_bram_mask;
      mask TypeOptions arith_type: Unsigned | Signed  (2's comp)
      mask TypeOptions data_width: 8 | 16 | 32 | 64 | 128
      mask TypeOptions optimization: Minimum_Area | Low_Power
  spec1_3 : Subsystem  Tag=xps:bram  AncestorBlock=xps_library/Shared_BRAM  mask{arith_type=Unsigned, addr_width=9, data_width=64, reg_prim_output=on, reg_core_output=on, optimization=Minimum_Area, data_bin_pt=0, init_vals=[0:2^10-1], sample_rate=1}
      mask prompts: arith_type "Output Data Type"; addr_width "Address width"; data_width "Data Width"; reg_prim_output "Register Primitive Output"; reg_core_output "Register Core Output"; data_bin_pt "Data Binary Point"; init_vals "Initial values (simulation only)"; sample_rate "Sample rate"
      mask init:
      | shared_bram_mask;
      mask TypeOptions arith_type: Unsigned | Signed  (2's comp)
      mask TypeOptions data_width: 8 | 16 | 32 | 64 | 128
      mask TypeOptions optimization: Minimum_Area | Low_Power
  sync_gen : Subsystem  AncestorBlock=casper_library_misc/sync_gen  mask(sync_gen){sim_acc_len=1, fft_size=2^7, fft_simult_inputs=8, pfb_fir_taps=4, reorder_vec=[2 2 2], scale=1}
      mask prompts: sim_acc_len "Simulation Accumulation Length"; fft_size "FFT Size"; fft_simult_inputs "Simultaneous Inputs (FFT)"; pfb_fir_taps "Taps in pfb_fir (use 1 if no pfb_fir)"; reorder_vec "Reorder Orders (e.g. [2 2 2])"
      mask help:
      | This block computes the sync period based on system parameters as
      | described in Casper memo.  Detailed descritions of the block's
      | variables can be found in the 'Block Documentation' section of
      | the CASPER wiki.
      mask init:
      | sync_gen_init(gcb, ...
      |     'sim_acc_len', sim_acc_len, ...
      |     'fft_size', fft_size, ...
      |     'fft_simult_inputs', fft_simult_inputs,...
      |     'pfb_fir_taps', pfb_fir_taps, ...
      |     'reorder_vec', reorder_vec, ...
      |     'scale', scale);
      settings: AttributesFormatString=sim_sync_period=128
      mask Help:
      | SyncPeriod=LCM(reorder_vec)*(acc_num)*(pfb_fir_len)*(fft_size/fft_simult_inputs)
      | 
      | See CASPER sync pulse memo for more details.
  sync_tree : Subsystem
  theta0 : Subsystem  Tag=xps:sw_reg  AncestorBlock=xps_library/software_register  mask(swreg){io_dir=From Processor, io_delay=0, sample_period=1, names=reg, bitwidths=32, bin_pts=0, arith_types=0, sim_port=off, show_format=on}
      mask prompts: io_dir "I/O direction"; io_delay "I/O delay"; sample_period "Sample period"; names "Bitfield names [msb...lsb]"; bitwidths "Bitfield widths"; bin_pts "Bitfield binary pts"; arith_types "Bitfield types, ufix=0, fix=1, bool=2"; sim_port "Provide sim input/output?"; show_format "Print format string?"
      mask help: A 32-bit software-accessible register. Can be divided into bitfields of varying widths and types using the fields in the block mask.
      mask init:
      | try
      |     swreg_init(gcb)
      | catch ex
      |     disp(sprintf('%s: %s', gcb, ex.message))
      |     errordlg(ex.message)
      | end
      settings: AttributesFormatString=1input:uf32.0 = 32 bits
      mask TypeOptions io_dir: To Processor | From Processor
      mask Callback io_dir:
      | mask_enables = get_param(gcb, 'MaskEnables');
      | mask_names = get_param(gcb, 'MaskNames');
      | if strcmp(get_param(gcb, 'io_dir'), 'To Processor'),
      |     mask_enables{ismember(mask_names, 'sample_period')} = 'off';
      | else
      |     mask_enables{ismember(mask_names, 'sample_period')} = 'on';
      | end
      | set_param(gcb, 'MaskEnables', mask_enables);
  theta1 : Subsystem  Tag=xps:sw_reg  AncestorBlock=xps_library/software_register  mask(swreg){io_dir=From Processor, io_delay=0, sample_period=1, names=reg, bitwidths=32, bin_pts=0, arith_types=0, sim_port=off, show_format=on}
      mask prompts: io_dir "I/O direction"; io_delay "I/O delay"; sample_period "Sample period"; names "Bitfield names [msb...lsb]"; bitwidths "Bitfield widths"; bin_pts "Bitfield binary pts"; arith_types "Bitfield types, ufix=0, fix=1, bool=2"; sim_port "Provide sim input/output?"; show_format "Print format string?"
      mask help: A 32-bit software-accessible register. Can be divided into bitfields of varying widths and types using the fields in the block mask.
      mask init:
      | try
      |     swreg_init(gcb)
      | catch ex
      |     disp(sprintf('%s: %s', gcb, ex.message))
      |     errordlg(ex.message)
      | end
      settings: AttributesFormatString=1input:uf32.0 = 32 bits
      mask TypeOptions io_dir: To Processor | From Processor
      mask Callback io_dir:
      | mask_enables = get_param(gcb, 'MaskEnables');
      | mask_names = get_param(gcb, 'MaskNames');
      | if strcmp(get_param(gcb, 'io_dir'), 'To Processor'),
      |     mask_enables{ismember(mask_names, 'sample_period')} = 'off';
      | else
      |     mask_enables{ismember(mask_names, 'sample_period')} = 'on';
      | end
      | set_param(gcb, 'MaskEnables', mask_enables);
  theta10 : Subsystem  Tag=xps:sw_reg  AncestorBlock=xps_library/software_register  mask(swreg){io_dir=From Processor, io_delay=0, sample_period=1, names=reg, bitwidths=32, bin_pts=0, arith_types=0, sim_port=off, show_format=on}
      mask prompts: io_dir "I/O direction"; io_delay "I/O delay"; sample_period "Sample period"; names "Bitfield names [msb...lsb]"; bitwidths "Bitfield widths"; bin_pts "Bitfield binary pts"; arith_types "Bitfield types, ufix=0, fix=1, bool=2"; sim_port "Provide sim input/output?"; show_format "Print format string?"
      mask help: A 32-bit software-accessible register. Can be divided into bitfields of varying widths and types using the fields in the block mask.
      mask init:
      | try
      |     swreg_init(gcb)
      | catch ex
      |     disp(sprintf('%s: %s', gcb, ex.message))
      |     errordlg(ex.message)
      | end
      settings: AttributesFormatString=1input:uf32.0 = 32 bits
      mask TypeOptions io_dir: To Processor | From Processor
      mask Callback io_dir:
      | mask_enables = get_param(gcb, 'MaskEnables');
      | mask_names = get_param(gcb, 'MaskNames');
      | if strcmp(get_param(gcb, 'io_dir'), 'To Processor'),
      |     mask_enables{ismember(mask_names, 'sample_period')} = 'off';
      | else
      |     mask_enables{ismember(mask_names, 'sample_period')} = 'on';
      | end
      | set_param(gcb, 'MaskEnables', mask_enables);
  theta2 : Subsystem  Tag=xps:sw_reg  AncestorBlock=xps_library/software_register  mask(swreg){io_dir=From Processor, io_delay=0, sample_period=1, names=reg, bitwidths=32, bin_pts=0, arith_types=0, sim_port=off, show_format=on}
      mask prompts: io_dir "I/O direction"; io_delay "I/O delay"; sample_period "Sample period"; names "Bitfield names [msb...lsb]"; bitwidths "Bitfield widths"; bin_pts "Bitfield binary pts"; arith_types "Bitfield types, ufix=0, fix=1, bool=2"; sim_port "Provide sim input/output?"; show_format "Print format string?"
      mask help: A 32-bit software-accessible register. Can be divided into bitfields of varying widths and types using the fields in the block mask.
      mask init:
      | try
      |     swreg_init(gcb)
      | catch ex
      |     disp(sprintf('%s: %s', gcb, ex.message))
      |     errordlg(ex.message)
      | end
      settings: AttributesFormatString=1input:uf32.0 = 32 bits
      mask TypeOptions io_dir: To Processor | From Processor
      mask Callback io_dir:
      | mask_enables = get_param(gcb, 'MaskEnables');
      | mask_names = get_param(gcb, 'MaskNames');
      | if strcmp(get_param(gcb, 'io_dir'), 'To Processor'),
      |     mask_enables{ismember(mask_names, 'sample_period')} = 'off';
      | else
      |     mask_enables{ismember(mask_names, 'sample_period')} = 'on';
      | end
      | set_param(gcb, 'MaskEnables', mask_enables);
  theta3 : Subsystem  Tag=xps:sw_reg  AncestorBlock=xps_library/software_register  mask(swreg){io_dir=From Processor, io_delay=0, sample_period=1, names=reg, bitwidths=32, bin_pts=0, arith_types=0, sim_port=off, show_format=on}
      mask prompts: io_dir "I/O direction"; io_delay "I/O delay"; sample_period "Sample period"; names "Bitfield names [msb...lsb]"; bitwidths "Bitfield widths"; bin_pts "Bitfield binary pts"; arith_types "Bitfield types, ufix=0, fix=1, bool=2"; sim_port "Provide sim input/output?"; show_format "Print format string?"
      mask help: A 32-bit software-accessible register. Can be divided into bitfields of varying widths and types using the fields in the block mask.
      mask init:
      | try
      |     swreg_init(gcb)
      | catch ex
      |     disp(sprintf('%s: %s', gcb, ex.message))
      |     errordlg(ex.message)
      | end
      settings: AttributesFormatString=1input:uf32.0 = 32 bits
      mask TypeOptions io_dir: To Processor | From Processor
      mask Callback io_dir:
      | mask_enables = get_param(gcb, 'MaskEnables');
      | mask_names = get_param(gcb, 'MaskNames');
      | if strcmp(get_param(gcb, 'io_dir'), 'To Processor'),
      |     mask_enables{ismember(mask_names, 'sample_period')} = 'off';
      | else
      |     mask_enables{ismember(mask_names, 'sample_period')} = 'on';
      | end
      | set_param(gcb, 'MaskEnables', mask_enables);
  theta4 : Subsystem  Tag=xps:sw_reg  AncestorBlock=xps_library/software_register  mask(swreg){io_dir=From Processor, io_delay=0, sample_period=1, names=reg, bitwidths=32, bin_pts=0, arith_types=0, sim_port=off, show_format=on}
      mask prompts: io_dir "I/O direction"; io_delay "I/O delay"; sample_period "Sample period"; names "Bitfield names [msb...lsb]"; bitwidths "Bitfield widths"; bin_pts "Bitfield binary pts"; arith_types "Bitfield types, ufix=0, fix=1, bool=2"; sim_port "Provide sim input/output?"; show_format "Print format string?"
      mask help: A 32-bit software-accessible register. Can be divided into bitfields of varying widths and types using the fields in the block mask.
      mask init:
      | try
      |     swreg_init(gcb)
      | catch ex
      |     disp(sprintf('%s: %s', gcb, ex.message))
      |     errordlg(ex.message)
      | end
      settings: AttributesFormatString=1input:uf32.0 = 32 bits
      mask TypeOptions io_dir: To Processor | From Processor
      mask Callback io_dir:
      | mask_enables = get_param(gcb, 'MaskEnables');
      | mask_names = get_param(gcb, 'MaskNames');
      | if strcmp(get_param(gcb, 'io_dir'), 'To Processor'),
      |     mask_enables{ismember(mask_names, 'sample_period')} = 'off';
      | else
      |     mask_enables{ismember(mask_names, 'sample_period')} = 'on';
      | end
      | set_param(gcb, 'MaskEnables', mask_enables);
  theta5 : Subsystem  Tag=xps:sw_reg  AncestorBlock=xps_library/software_register  mask(swreg){io_dir=From Processor, io_delay=0, sample_period=1, names=reg, bitwidths=32, bin_pts=0, arith_types=0, sim_port=off, show_format=on}
      mask prompts: io_dir "I/O direction"; io_delay "I/O delay"; sample_period "Sample period"; names "Bitfield names [msb...lsb]"; bitwidths "Bitfield widths"; bin_pts "Bitfield binary pts"; arith_types "Bitfield types, ufix=0, fix=1, bool=2"; sim_port "Provide sim input/output?"; show_format "Print format string?"
      mask help: A 32-bit software-accessible register. Can be divided into bitfields of varying widths and types using the fields in the block mask.
      mask init:
      | try
      |     swreg_init(gcb)
      | catch ex
      |     disp(sprintf('%s: %s', gcb, ex.message))
      |     errordlg(ex.message)
      | end
      settings: AttributesFormatString=1input:uf32.0 = 32 bits
      mask TypeOptions io_dir: To Processor | From Processor
      mask Callback io_dir:
      | mask_enables = get_param(gcb, 'MaskEnables');
      | mask_names = get_param(gcb, 'MaskNames');
      | if strcmp(get_param(gcb, 'io_dir'), 'To Processor'),
      |     mask_enables{ismember(mask_names, 'sample_period')} = 'off';
      | else
      |     mask_enables{ismember(mask_names, 'sample_period')} = 'on';
      | end
      | set_param(gcb, 'MaskEnables', mask_enables);
  theta6 : Subsystem  Tag=xps:sw_reg  AncestorBlock=xps_library/software_register  mask(swreg){io_dir=From Processor, io_delay=0, sample_period=1, names=reg, bitwidths=32, bin_pts=0, arith_types=0, sim_port=off, show_format=on}
      mask prompts: io_dir "I/O direction"; io_delay "I/O delay"; sample_period "Sample period"; names "Bitfield names [msb...lsb]"; bitwidths "Bitfield widths"; bin_pts "Bitfield binary pts"; arith_types "Bitfield types, ufix=0, fix=1, bool=2"; sim_port "Provide sim input/output?"; show_format "Print format string?"
      mask help: A 32-bit software-accessible register. Can be divided into bitfields of varying widths and types using the fields in the block mask.
      mask init:
      | try
      |     swreg_init(gcb)
      | catch ex
      |     disp(sprintf('%s: %s', gcb, ex.message))
      |     errordlg(ex.message)
      | end
      settings: AttributesFormatString=1input:uf32.0 = 32 bits
      mask TypeOptions io_dir: To Processor | From Processor
      mask Callback io_dir:
      | mask_enables = get_param(gcb, 'MaskEnables');
      | mask_names = get_param(gcb, 'MaskNames');
      | if strcmp(get_param(gcb, 'io_dir'), 'To Processor'),
      |     mask_enables{ismember(mask_names, 'sample_period')} = 'off';
      | else
      |     mask_enables{ismember(mask_names, 'sample_period')} = 'on';
      | end
      | set_param(gcb, 'MaskEnables', mask_enables);
  theta7 : Subsystem  Tag=xps:sw_reg  AncestorBlock=xps_library/software_register  mask(swreg){io_dir=From Processor, io_delay=0, sample_period=1, names=reg, bitwidths=32, bin_pts=0, arith_types=0, sim_port=off, show_format=on}
      mask prompts: io_dir "I/O direction"; io_delay "I/O delay"; sample_period "Sample period"; names "Bitfield names [msb...lsb]"; bitwidths "Bitfield widths"; bin_pts "Bitfield binary pts"; arith_types "Bitfield types, ufix=0, fix=1, bool=2"; sim_port "Provide sim input/output?"; show_format "Print format string?"
      mask help: A 32-bit software-accessible register. Can be divided into bitfields of varying widths and types using the fields in the block mask.
      mask init:
      | try
      |     swreg_init(gcb)
      | catch ex
      |     disp(sprintf('%s: %s', gcb, ex.message))
      |     errordlg(ex.message)
      | end
      settings: AttributesFormatString=1input:uf32.0 = 32 bits
      mask TypeOptions io_dir: To Processor | From Processor
      mask Callback io_dir:
      | mask_enables = get_param(gcb, 'MaskEnables');
      | mask_names = get_param(gcb, 'MaskNames');
      | if strcmp(get_param(gcb, 'io_dir'), 'To Processor'),
      |     mask_enables{ismember(mask_names, 'sample_period')} = 'off';
      | else
      |     mask_enables{ismember(mask_names, 'sample_period')} = 'on';
      | end
      | set_param(gcb, 'MaskEnables', mask_enables);
  theta8 : Subsystem  Tag=xps:sw_reg  AncestorBlock=xps_library/software_register  mask(swreg){io_dir=From Processor, io_delay=0, sample_period=1, names=reg, bitwidths=32, bin_pts=0, arith_types=0, sim_port=off, show_format=on}
      mask prompts: io_dir "I/O direction"; io_delay "I/O delay"; sample_period "Sample period"; names "Bitfield names [msb...lsb]"; bitwidths "Bitfield widths"; bin_pts "Bitfield binary pts"; arith_types "Bitfield types, ufix=0, fix=1, bool=2"; sim_port "Provide sim input/output?"; show_format "Print format string?"
      mask help: A 32-bit software-accessible register. Can be divided into bitfields of varying widths and types using the fields in the block mask.
      mask init:
      | try
      |     swreg_init(gcb)
      | catch ex
      |     disp(sprintf('%s: %s', gcb, ex.message))
      |     errordlg(ex.message)
      | end
      settings: AttributesFormatString=1input:uf32.0 = 32 bits
      mask TypeOptions io_dir: To Processor | From Processor
      mask Callback io_dir:
      | mask_enables = get_param(gcb, 'MaskEnables');
      | mask_names = get_param(gcb, 'MaskNames');
      | if strcmp(get_param(gcb, 'io_dir'), 'To Processor'),
      |     mask_enables{ismember(mask_names, 'sample_period')} = 'off';
      | else
      |     mask_enables{ismember(mask_names, 'sample_period')} = 'on';
      | end
      | set_param(gcb, 'MaskEnables', mask_enables);
  theta9 : Subsystem  Tag=xps:sw_reg  AncestorBlock=xps_library/software_register  mask(swreg){io_dir=From Processor, io_delay=0, sample_period=1, names=reg, bitwidths=32, bin_pts=0, arith_types=0, sim_port=off, show_format=on}
      mask prompts: io_dir "I/O direction"; io_delay "I/O delay"; sample_period "Sample period"; names "Bitfield names [msb...lsb]"; bitwidths "Bitfield widths"; bin_pts "Bitfield binary pts"; arith_types "Bitfield types, ufix=0, fix=1, bool=2"; sim_port "Provide sim input/output?"; show_format "Print format string?"
      mask help: A 32-bit software-accessible register. Can be divided into bitfields of varying widths and types using the fields in the block mask.
      mask init:
      | try
      |     swreg_init(gcb)
      | catch ex
      |     disp(sprintf('%s: %s', gcb, ex.message))
      |     errordlg(ex.message)
      | end
      settings: AttributesFormatString=1input:uf32.0 = 32 bits
      mask TypeOptions io_dir: To Processor | From Processor
      mask Callback io_dir:
      | mask_enables = get_param(gcb, 'MaskEnables');
      | mask_names = get_param(gcb, 'MaskNames');
      | if strcmp(get_param(gcb, 'io_dir'), 'To Processor'),
      |     mask_enables{ismember(mask_names, 'sample_period')} = 'off';
      | else
      |     mask_enables{ismember(mask_names, 'sample_period')} = 'on';
      | end
      | set_param(gcb, 'MaskEnables', mask_enables);
  wires:
  sync_gen/1(sync_out) -> Delay11/1
  Delay11/1 -> [sync_gen]
  [sync_gen] -> pipeline9/1(d)
  Constant3/1 -> acc_len1/1(sim_1)
  acc_len1/1(in_reg) -> pipeline31/1(d)
  pipeline31/1(q) -> [acc_len1]
  Constant4/1 -> cnt_rst/1(sim_1)
  cnt_rst/1(in_reg) -> pipeline32/1(d)
  pipeline32/1(q) -> Slice/1
  Slice/1 -> [cnt_rst]
  Delay2/1 -> Delay3/1
  Delay17/1 -> power1/1
  Delay12/1 -> acc_cntrl/2(sync)
  [acc_len1] -> acc_cntrl/1(acc_len)
  [cnt_rst] -> acc_cntrl/3(rst)
  Delay13/1 -> pipeline36/1(d)
  pipeline19/1(q) -> simple_bram_vacc3/1(new_acc)
  pipeline17/1(q) -> simple_bram_vacc2/1(new_acc)
  pipeline15/1(q) -> simple_bram_vacc1/1(new_acc)
  pipeline22/1(q) -> simple_bram_vacc/1(new_acc)
  pipeline13/1(q) -> simple_bram_vacc/2(din)
  pipeline14/1(q) -> simple_bram_vacc1/2(din)
  pipeline16/1(q) -> simple_bram_vacc2/2(din)
  pipeline18/1(q) -> simple_bram_vacc3/2(din)
  pipeline20/1(q) -> Counter21/1
  simple_bram_vacc/2(valid) -> Counter21/2, pipeline23/1(d)
  simple_bram_vacc/1(dout) -> Reinterpret/1
  simple_bram_vacc1/1(dout) -> Reinterpret1/1
  simple_bram_vacc2/1(dout) -> Reinterpret2/1
  simple_bram_vacc3/1(dout) -> Reinterpret3/1
  Reinterpret/1 -> pipeline21/1(d)
  Reinterpret1/1 -> pipeline24/1(d)
  Reinterpret2/1 -> pipeline26/1(d)
  Reinterpret3/1 -> pipeline29/1(d)
  Counter21/1 -> Relational1/2, Relational2/2
  Constant12/1 -> Mux2/2
  Constant5/1 -> Mux1/2
  Constant6/1 -> Mux3/2
  Constant7/1 -> Mux4/2
  edge_detect/1 -> Accumulator/2, Logical1/1
  adder_tree/1(sync_out) -> Accumulator/3, edge_detect/1
  adder_tree/2(dout) -> Accumulator/1
  Register/1 -> [frb_detector_1]
  [cnt_rst] -> Register/2
  Relational/1 -> Register/3, Register/1
  simple_bram_vacc3/2(valid) -> Terminator21/1
  pipeline23/1(q) -> Mux4/1, Mux3/1, Mux1/1, Parallel_Dedispersor_v11/1(Valid), pipeline67/1(d), Logical2/1
  pipeline67/1(q) -> pipeline41/1(d)
  Accumulator/1 -> Relational/2, ACC1/2(data_in)
  Counter1/1 -> ACC1/1(addr)
  ACC1/1(data_out) -> Terminator22/1
  Logical1/1 -> Counter1/1
  pipeline9/1(q) -> pfb_fir_real/1(sync)
  asiaa_adc5g/17(sync_out) -> Terminator2/1
  asiaa_adc5g/1(a0) -> conv_bus0/1(i0)
  asiaa_adc5g/2(a1) -> conv_bus0/2(i1)
  asiaa_adc5g/3(a2) -> conv_bus0/3(i2)
  asiaa_adc5g/4(a3) -> conv_bus0/4(i3)
  asiaa_adc5g/5(a4) -> conv_bus0/5(i4)
  asiaa_adc5g/6(a5) -> conv_bus0/6(i5)
  asiaa_adc5g/7(a6) -> conv_bus0/7(i6)
  asiaa_adc5g/8(a7) -> conv_bus0/8(i7)
  conv_bus0/1(q0) -> pipeline301/1
  conv_bus0/2(q1) -> pipeline349/1
  conv_bus0/3(q2) -> pipeline399/1
  conv_bus0/4(q3) -> pipeline400/1
  conv_bus0/5(q4) -> pipeline401/1
  conv_bus0/6(q5) -> pipeline402/1
  conv_bus0/7(q6) -> pipeline300/1
  conv_bus0/8(q7) -> pipeline299/1
  pipeline3/1(q) -> pfb_fir_real/4(pol1_in3)
  pipeline5/1(q) -> pfb_fir_real/6(pol1_in5)
  pipeline1/1(q) -> pfb_fir_real/2(pol1_in1)
  pipeline2/1(q) -> pfb_fir_real/3(pol1_in2)
  pipeline4/1(q) -> pfb_fir_real/5(pol1_in4)
  pipeline6/1(q) -> pfb_fir_real/7(pol1_in6)
  pipeline7/1(q) -> pfb_fir_real/8(pol1_in7)
  pipeline8/1(q) -> pfb_fir_real/9(pol1_in8)
  Delay6/1 -> fft_wideband_real/1(sync)
  pfb_fir_real/1(sync_out) -> Delay6/1
  Constant/1 -> fft_wideband_real/2(shift)
  pfb_fir_real/2(pol1_out1) -> Delay1/1
  pfb_fir_real/3(pol1_out2) -> Delay4/1
  pfb_fir_real/4(pol1_out3) -> Delay7/1
  pfb_fir_real/5(pol1_out4) -> Delay9/1
  pfb_fir_real/6(pol1_out5) -> Delay16/1
  pfb_fir_real/7(pol1_out6) -> Delay20/1
  pfb_fir_real/8(pol1_out7) -> Delay22/1
  pfb_fir_real/9(pol1_out8) -> Delay23/1
  Delay23/1 -> fft_wideband_real/10(in07)
  Delay16/1 -> fft_wideband_real/7(in04)
  Delay9/1 -> fft_wideband_real/6(in03)
  Delay20/1 -> fft_wideband_real/8(in05)
  Delay7/1 -> fft_wideband_real/5(in02)
  Delay1/1 -> fft_wideband_real/3(in00)
  Delay22/1 -> fft_wideband_real/9(in06)
  Delay4/1 -> fft_wideband_real/4(in01)
  fft_wideband_real/6(of) -> Terminator3/1
  fft_wideband_real/1(sync_out) -> Delay2/1
  Delay34/1 -> power2/1
  Delay33/1 -> pipeline33/1(d)
  Delay36/1 -> power3/1
  Delay35/1 -> pipeline34/1(d)
  Delay38/1 -> power4/1
  Delay37/1 -> pipeline35/1(d)
  fft_wideband_real/2(out00) -> Delay17/1
  fft_wideband_real/3(out01) -> Delay34/1
  fft_wideband_real/4(out02) -> Delay36/1
  fft_wideband_real/5(out03) -> Delay38/1
  acc_cntrl/1(new_acc) -> pipeline98/1(d)
  pipeline36/1(q) -> pipeline111/1(d)
  pipeline33/1(q) -> pipeline113/1(d)
  pipeline34/1(q) -> pipeline143/1(d)
  pipeline35/1(q) -> pipeline145/1(d)
  pipeline21/1(q) -> Mux2/3
  pipeline24/1(q) -> Mux1/3
  pipeline26/1(q) -> Mux3/3
  pipeline29/1(q) -> Mux4/3
  Mux2/1 -> Parallel_Dedispersor_v11/2(Data1)
  Mux1/1 -> Parallel_Dedispersor_v11/3(Data2)
  Mux3/1 -> Parallel_Dedispersor_v11/4(Data3)
  Mux4/1 -> Parallel_Dedispersor_v11/5(Data4)
  Parallel_Dedispersor_v11/1(Out1) -> pipeline86/1(d)
  Parallel_Dedispersor_v11/2(Out2) -> pipeline87/1(d)
  Parallel_Dedispersor_v11/3(Out3) -> pipeline88/1(d)
  Parallel_Dedispersor_v11/4(Out4) -> pipeline89/1(d)
  pipeline86/1(q) -> adder_tree/2(din1)
  pipeline87/1(q) -> adder_tree/3(din2)
  pipeline88/1(q) -> adder_tree/4(din3)
  pipeline89/1(q) -> adder_tree/5(din4)
  pipeline109/1(q) -> Logical2/3
  pipeline108/1(q) -> Logical2/2
  Logical2/1 -> Mux2/1
  Relational1/1 -> pipeline108/1(d)
  Relational2/1 -> pipeline109/1(d)
  Constant11/1 -> Relational1/1
  Constant13/1 -> Relational2/1
  Constant14/1 -> Logical1/2
  theta1/1(in_reg) -> Convert1/1
  Convert1/1 -> Relational/1
  Constant26/1 -> acc_len2/1(sim_1)
  acc_len2/1(in_reg) -> pipeline134/1(d)
  pipeline134/1(q) -> [acc_len2]
  Constant27/1 -> acc_len3/1(sim_1)
  acc_len3/1(in_reg) -> pipeline135/1(d)
  pipeline135/1(q) -> [acc_len3]
  Constant28/1 -> acc_len4/1(sim_1)
  acc_len4/1(in_reg) -> pipeline136/1(d)
  pipeline136/1(q) -> [acc_len4]
  Constant29/1 -> acc_len5/1(sim_1)
  acc_len5/1(in_reg) -> pipeline137/1(d)
  pipeline137/1(q) -> [acc_len5]
  Constant30/1 -> acc_len6/1(sim_1)
  acc_len6/1(in_reg) -> pipeline138/1(d)
  pipeline138/1(q) -> [acc_len6]
  Constant31/1 -> acc_len7/1(sim_1)
  acc_len7/1(in_reg) -> pipeline139/1(d)
  pipeline139/1(q) -> [acc_len7]
  Constant87/1 -> acc_len8/1(sim_1)
  acc_len8/1(in_reg) -> pipeline425/1(d)
  pipeline425/1(q) -> [acc_len8]
  Constant88/1 -> acc_len9/1(sim_1)
  acc_len9/1(in_reg) -> pipeline426/1(d)
  pipeline426/1(q) -> [acc_len9]
  Constant89/1 -> acc_len10/1(sim_1)
  acc_len10/1(in_reg) -> pipeline427/1(d)
  pipeline427/1(q) -> [acc_len10]
  bus_create0/1(bus_out) -> pipeline599/1(d)
  Constant123/1 -> adcsnap0/3(trig), adcsnap0/2(we)
  pipeline599/1(q) -> adcsnap0/1(din)
  Delay127/1 -> acc_cntrl10/2(sync)
  [acc_len] -> acc_cntrl10/1(acc_len)
  [cnt_rst] -> acc_cntrl10/3(rst)
  Constant124/1 -> acc_len/1(sim_1)
  acc_len/1(in_reg) -> pipeline600/1(d)
  pipeline600/1(q) -> [acc_len]
  Delay119/1 -> pipeline602/1(d)
  pipeline625/1(q) -> simple_bram_vacc86/1(new_acc)
  pipeline617/1(q) -> simple_bram_vacc86/2(din)
  pipeline624/1(q) -> Counter20/1
  acc_cntrl10/1(new_acc) -> pipeline393/1(d)
  pipeline602/1(q) -> pipeline389/1(d)
  simple_bram_vacc86/1(dout) -> Reinterpret80/1
  spec0_0/1(data_out) -> Terminator90/1
  Reinterpret80/1 -> Convert12/1
  simple_bram_vacc86/2(valid) -> Counter20/2, spec0_0/3(we)
  pipeline603/1(q) -> simple_bram_vacc40/1(new_acc)
  pipeline601/1(q) -> simple_bram_vacc40/2(din)
  simple_bram_vacc40/1(dout) -> Reinterpret81/1
  spec0_1/1(data_out) -> Terminator83/1
  Reinterpret81/1 -> Convert13/1
  simple_bram_vacc40/2(valid) -> spec0_1/3(we)
  pipeline607/1(q) -> simple_bram_vacc42/1(new_acc)
  pipeline606/1(q) -> simple_bram_vacc42/2(din)
  simple_bram_vacc42/1(dout) -> Reinterpret82/1
  spec0_2/1(data_out) -> Terminator85/1
  Reinterpret82/1 -> Convert14/1
  simple_bram_vacc42/2(valid) -> spec0_2/3(we)
  pipeline605/1(q) -> simple_bram_vacc41/1(new_acc)
  pipeline604/1(q) -> simple_bram_vacc41/2(din)
  simple_bram_vacc41/1(dout) -> Reinterpret83/1
  spec0_3/1(data_out) -> Terminator84/1
  Reinterpret83/1 -> Convert15/1
  simple_bram_vacc41/2(valid) -> spec0_3/3(we)
  Counter20/1 -> spec0_1/1(addr), spec0_3/1(addr), spec0_2/1(addr), spec0_0/1(addr)
  Delay120/1 -> pipeline616/1(d)
  pipeline616/1(q) -> pipeline390/1(d)
  Delay121/1 -> pipeline618/1(d)
  pipeline618/1(q) -> pipeline391/1(d)
  Delay122/1 -> pipeline619/1(d)
  pipeline619/1(q) -> pipeline392/1(d)
  asiaa_adc5g/16(c7) -> Terminator91/1
  asiaa_adc5g/15(c6) -> Terminator92/1
  asiaa_adc5g/14(c5) -> Terminator93/1
  asiaa_adc5g/13(c4) -> Terminator94/1
  asiaa_adc5g/12(c3) -> Terminator95/1
  asiaa_adc5g/11(c2) -> Terminator96/1
  asiaa_adc5g/10(c1) -> Terminator97/1
  asiaa_adc5g/9(c0) -> Terminator98/1
  Constant80/1 -> asiaa_adc5g/2(sim_c)
  Constant1/1 -> asiaa_adc5g/3(sim_sync)
  simple_bram_vacc1/2(valid) -> Terminator18/1
  simple_bram_vacc2/2(valid) -> Terminator1/1
  Constant81/1 -> asiaa_adc5g/1(sim_a)
  Delay5/1 -> acc_cntrl1/2(sync)
  [acc_len2] -> acc_cntrl1/1(acc_len)
  [cnt_rst] -> acc_cntrl1/3(rst)
  Delay8/1 -> pipeline52/1(d)
  pipeline39/1(q) -> simple_bram_vacc7/1(new_acc)
  pipeline30/1(q) -> simple_bram_vacc6/1(new_acc)
  pipeline27/1(q) -> simple_bram_vacc5/1(new_acc)
  pipeline44/1(q) -> simple_bram_vacc4/1(new_acc)
  pipeline12/1(q) -> simple_bram_vacc4/2(din)
  pipeline25/1(q) -> simple_bram_vacc5/2(din)
  pipeline28/1(q) -> simple_bram_vacc6/2(din)
  pipeline38/1(q) -> simple_bram_vacc7/2(din)
  pipeline40/1(q) -> Counter3/1
  simple_bram_vacc4/2(valid) -> pipeline45/1(d), Counter3/2
  simple_bram_vacc4/1(dout) -> Reinterpret4/1
  simple_bram_vacc5/1(dout) -> Reinterpret5/1
  simple_bram_vacc6/1(dout) -> Reinterpret6/1
  simple_bram_vacc7/1(dout) -> Reinterpret7/1
  Reinterpret4/1 -> pipeline43/1(d)
  Reinterpret5/1 -> pipeline46/1(d)
  Reinterpret6/1 -> pipeline47/1(d)
  Reinterpret7/1 -> pipeline48/1(d)
  Counter3/1 -> Relational5/2, Relational4/2
  Constant8/1 -> Mux6/2
  Constant15/1 -> Mux5/2
  Constant16/1 -> Mux7/2
  Constant17/1 -> Mux8/2
  simple_bram_vacc7/2(valid) -> Terminator6/1
  pipeline45/1(q) -> Mux8/1, Mux7/1, Mux5/1, Parallel_Dedispersor_v1/1(Valid), pipeline56/1(d), Logical4/1
  pipeline56/1(q) -> pipeline54/1(d)
  Delay10/1 -> pipeline49/1(d)
  Delay14/1 -> pipeline50/1(d)
  Delay15/1 -> pipeline51/1(d)
  acc_cntrl1/1(new_acc) -> pipeline93/1(d)
  pipeline52/1(q) -> pipeline179/1(d)
  pipeline49/1(q) -> pipeline184/1(d)
  pipeline50/1(q) -> pipeline195/1(d)
  pipeline51/1(q) -> pipeline197/1(d)
  pipeline43/1(q) -> Mux6/3
  pipeline46/1(q) -> Mux5/3
  pipeline47/1(q) -> Mux7/3
  pipeline48/1(q) -> Mux8/3
  Mux6/1 -> Parallel_Dedispersor_v1/2(Data1)
  Mux5/1 -> Parallel_Dedispersor_v1/3(Data2)
  Mux7/1 -> Parallel_Dedispersor_v1/4(Data3)
  Mux8/1 -> Parallel_Dedispersor_v1/5(Data4)
  Parallel_Dedispersor_v1/1(Out1) -> pipeline57/1(d)
  Parallel_Dedispersor_v1/2(Out2) -> pipeline58/1(d)
  Parallel_Dedispersor_v1/3(Out3) -> pipeline59/1(d)
  Parallel_Dedispersor_v1/4(Out4) -> pipeline60/1(d)
  pipeline11/1(q) -> Logical4/3
  pipeline10/1(q) -> Logical4/2
  Logical4/1 -> Mux6/1
  Relational4/1 -> pipeline10/1(d)
  Relational5/1 -> pipeline11/1(d)
  Constant2/1 -> Relational4/1
  Constant9/1 -> Relational5/1
  simple_bram_vacc5/2(valid) -> Terminator5/1
  simple_bram_vacc6/2(valid) -> Terminator4/1
  Delay19/1 -> acc_cntrl2/2(sync)
  [acc_len3] -> acc_cntrl2/1(acc_len)
  [cnt_rst] -> acc_cntrl2/3(rst)
  Delay21/1 -> pipeline92/1(d)
  pipeline73/1(q) -> simple_bram_vacc11/1(new_acc)
  pipeline71/1(q) -> simple_bram_vacc10/1(new_acc)
  pipeline69/1(q) -> simple_bram_vacc9/1(new_acc)
  pipeline76/1(q) -> simple_bram_vacc8/1(new_acc)
  pipeline66/1(q) -> simple_bram_vacc8/2(din)
  pipeline68/1(q) -> simple_bram_vacc9/2(din)
  pipeline70/1(q) -> simple_bram_vacc10/2(din)
  pipeline72/1(q) -> simple_bram_vacc11/2(din)
  pipeline74/1(q) -> Counter6/1
  simple_bram_vacc8/2(valid) -> pipeline77/1(d), Counter6/2
  simple_bram_vacc8/1(dout) -> Reinterpret8/1
  simple_bram_vacc9/1(dout) -> Reinterpret9/1
  simple_bram_vacc10/1(dout) -> Reinterpret10/1
  simple_bram_vacc11/1(dout) -> Reinterpret11/1
  Reinterpret8/1 -> pipeline75/1(d)
  Reinterpret9/1 -> pipeline78/1(d)
  Reinterpret10/1 -> pipeline80/1(d)
  Reinterpret11/1 -> pipeline83/1(d)
  Counter6/1 -> Relational8/2, Relational7/2
  Constant20/1 -> Mux10/2
  Constant33/1 -> Mux9/2
  Constant34/1 -> Mux11/2
  Constant35/1 -> Mux12/2
  simple_bram_vacc11/2(valid) -> Terminator10/1
  pipeline77/1(q) -> Mux12/1, Mux11/1, Mux9/1, Parallel_Dedispersor_v2/1(Valid), pipeline119/1(d), Logical6/1
  pipeline119/1(q) -> pipeline97/1(d)
  Delay26/1 -> pipeline85/1(d)
  Delay27/1 -> pipeline90/1(d)
  Delay28/1 -> pipeline91/1(d)
  acc_cntrl2/1(new_acc) -> pipeline291/1(d)
  pipeline92/1(q) -> pipeline235/1(d)
  pipeline85/1(q) -> pipeline240/1(d)
  pipeline90/1(q) -> pipeline251/1(d)
  pipeline91/1(q) -> pipeline253/1(d)
  pipeline75/1(q) -> Mux10/3
  pipeline78/1(q) -> Mux9/3
  pipeline80/1(q) -> Mux11/3
  pipeline83/1(q) -> Mux12/3
  Mux10/1 -> Parallel_Dedispersor_v2/2(Data1)
  Mux9/1 -> Parallel_Dedispersor_v2/3(Data2)
  Mux11/1 -> Parallel_Dedispersor_v2/4(Data3)
  Mux12/1 -> Parallel_Dedispersor_v2/5(Data4)
  Parallel_Dedispersor_v2/1(Out1) -> pipeline120/1(d)
  Parallel_Dedispersor_v2/2(Out2) -> pipeline121/1(d)
  Parallel_Dedispersor_v2/3(Out3) -> pipeline122/1(d)
  Parallel_Dedispersor_v2/4(Out4) -> pipeline123/1(d)
  pipeline63/1(q) -> Logical6/3
  pipeline62/1(q) -> Logical6/2
  Logical6/1 -> Mux10/1
  Relational7/1 -> pipeline62/1(d)
  Relational8/1 -> pipeline63/1(d)
  Constant19/1 -> Relational7/1
  Constant21/1 -> Relational8/1
  simple_bram_vacc9/2(valid) -> Terminator9/1
  simple_bram_vacc10/2(valid) -> Terminator8/1
  Delay29/1 -> acc_cntrl3/2(sync)
  [acc_len4] -> acc_cntrl3/1(acc_len)
  [cnt_rst] -> acc_cntrl3/3(rst)
  Delay30/1 -> pipeline110/1(d)
  pipeline95/1(q) -> simple_bram_vacc13/1(new_acc)
  pipeline84/1(q) -> simple_bram_vacc12/1(new_acc)
  pipeline81/1(q) -> simple_bram_vacc15/1(new_acc)
  pipeline100/1(q) -> simple_bram_vacc14/1(new_acc)
  pipeline65/1(q) -> simple_bram_vacc14/2(din)
  pipeline79/1(q) -> simple_bram_vacc15/2(din)
  pipeline82/1(q) -> simple_bram_vacc12/2(din)
  pipeline94/1(q) -> simple_bram_vacc13/2(din)
  pipeline96/1(q) -> Counter7/1
  simple_bram_vacc14/2(valid) -> Counter7/2, pipeline101/1(d)
  simple_bram_vacc14/1(dout) -> Reinterpret12/1
  simple_bram_vacc15/1(dout) -> Reinterpret13/1
  simple_bram_vacc12/1(dout) -> Reinterpret14/1
  simple_bram_vacc13/1(dout) -> Reinterpret15/1
  Reinterpret12/1 -> pipeline99/1(d)
  Reinterpret13/1 -> pipeline102/1(d)
  Reinterpret14/1 -> pipeline103/1(d)
  Reinterpret15/1 -> pipeline104/1(d)
  Counter7/1 -> Relational10/2, Relational11/2
  Constant36/1 -> Mux14/2
  Constant23/1 -> Mux13/2
  Constant24/1 -> Mux15/2
  Constant25/1 -> Mux16/2
  simple_bram_vacc13/2(valid) -> Terminator14/1
  pipeline101/1(q) -> Mux16/1, Mux15/1, Mux13/1, Parallel_Dedispersor_v3/1(Valid), pipeline114/1(d), Logical8/1
  pipeline114/1(q) -> pipeline112/1(d)
  Delay18/1 -> pipeline105/1(d)
  Delay24/1 -> pipeline106/1(d)
  Delay25/1 -> pipeline107/1(d)
  acc_cntrl3/1(new_acc) -> pipeline353/1(d)
  pipeline110/1(q) -> pipeline296/1(d)
  pipeline105/1(q) -> pipeline325/1(d)
  pipeline106/1(q) -> pipeline327/1(d)
  pipeline107/1(q) -> pipeline352/1(d)
  pipeline99/1(q) -> Mux14/3
  pipeline102/1(q) -> Mux13/3
  pipeline103/1(q) -> Mux15/3
  pipeline104/1(q) -> Mux16/3
  Mux14/1 -> Parallel_Dedispersor_v3/2(Data1)
  Mux13/1 -> Parallel_Dedispersor_v3/3(Data2)
  Mux15/1 -> Parallel_Dedispersor_v3/4(Data3)
  Mux16/1 -> Parallel_Dedispersor_v3/5(Data4)
  Parallel_Dedispersor_v3/1(Out1) -> pipeline115/1(d)
  Parallel_Dedispersor_v3/2(Out2) -> pipeline116/1(d)
  Parallel_Dedispersor_v3/3(Out3) -> pipeline117/1(d)
  Parallel_Dedispersor_v3/4(Out4) -> pipeline118/1(d)
  pipeline64/1(q) -> Logical8/3
  pipeline61/1(q) -> Logical8/2
  Logical8/1 -> Mux14/1
  Relational10/1 -> pipeline61/1(d)
  Relational11/1 -> pipeline64/1(d)
  Constant32/1 -> Relational10/1
  Constant37/1 -> Relational11/1
  simple_bram_vacc15/2(valid) -> Terminator13/1
  simple_bram_vacc12/2(valid) -> Terminator12/1
  Delay32/1 -> acc_cntrl4/2(sync)
  [acc_len5] -> acc_cntrl4/1(acc_len)
  [cnt_rst] -> acc_cntrl4/3(rst)
  Delay39/1 -> pipeline178/1(d)
  pipeline163/1(q) -> simple_bram_vacc17/1(new_acc)
  pipeline161/1(q) -> simple_bram_vacc16/1(new_acc)
  pipeline159/1(q) -> simple_bram_vacc25/1(new_acc)
  pipeline166/1(q) -> simple_bram_vacc24/1(new_acc)
  pipeline157/1(q) -> simple_bram_vacc24/2(din)
  pipeline158/1(q) -> simple_bram_vacc25/2(din)
  pipeline160/1(q) -> simple_bram_vacc16/2(din)
  pipeline162/1(q) -> simple_bram_vacc17/2(din)
  pipeline164/1(q) -> Counter10/1
  simple_bram_vacc24/2(valid) -> pipeline167/1(d), Counter10/2
  simple_bram_vacc24/1(dout) -> Reinterpret16/1
  simple_bram_vacc25/1(dout) -> Reinterpret17/1
  simple_bram_vacc16/1(dout) -> Reinterpret24/1
  simple_bram_vacc17/1(dout) -> Reinterpret25/1
  Reinterpret16/1 -> pipeline165/1(d)
  Reinterpret17/1 -> pipeline168/1(d)
  Reinterpret24/1 -> pipeline170/1(d)
  Reinterpret25/1 -> pipeline173/1(d)
  Counter10/1 -> Relational16/2, Relational13/2
  Constant40/1 -> Mux25/2
  Constant61/1 -> Mux17/2
  Constant62/1 -> Mux26/2
  Constant63/1 -> Mux27/2
  simple_bram_vacc17/2(valid) -> Terminator27/1
  pipeline167/1(q) -> Mux27/1, Mux26/1, Mux17/1, Parallel_Dedispersor_v4/1(Valid), pipeline209/1(d), Logical10/1
  pipeline209/1(q) -> pipeline183/1(d)
  Delay52/1 -> pipeline175/1(d)
  Delay53/1 -> pipeline176/1(d)
  Delay54/1 -> pipeline177/1(d)
  acc_cntrl4/1(new_acc) -> pipeline358/1(d)
  pipeline178/1(q) -> pipeline354/1(d)
  pipeline175/1(q) -> pipeline355/1(d)
  pipeline176/1(q) -> pipeline356/1(d)
  pipeline177/1(q) -> pipeline357/1(d)
  pipeline165/1(q) -> Mux25/3
  pipeline168/1(q) -> Mux17/3
  pipeline170/1(q) -> Mux26/3
  pipeline173/1(q) -> Mux27/3
  Mux25/1 -> Parallel_Dedispersor_v4/2(Data1)
  Mux17/1 -> Parallel_Dedispersor_v4/3(Data2)
  Mux26/1 -> Parallel_Dedispersor_v4/4(Data3)
  Mux27/1 -> Parallel_Dedispersor_v4/5(Data4)
  Parallel_Dedispersor_v4/1(Out1) -> pipeline228/1(d)
  Parallel_Dedispersor_v4/2(Out2) -> pipeline229/1(d)
  Parallel_Dedispersor_v4/3(Out3) -> pipeline230/1(d)
  Parallel_Dedispersor_v4/4(Out4) -> pipeline231/1(d)
  pipeline140/1(q) -> Logical10/3
  pipeline133/1(q) -> Logical10/2
  Logical10/1 -> Mux25/1
  Relational13/1 -> pipeline133/1(d)
  Relational16/1 -> pipeline140/1(d)
  Constant39/1 -> Relational13/1
  Constant41/1 -> Relational16/1
  Delay3/1 -> Delay68/1
  simple_bram_vacc25/2(valid) -> Terminator26/1
  simple_bram_vacc16/2(valid) -> Terminator16/1
  power4/1 -> Delay71/1
  power2/1 -> Delay69/1
  Delay55/1 -> acc_cntrl5/2(sync)
  [acc_len6] -> acc_cntrl5/1(acc_len)
  [cnt_rst] -> acc_cntrl5/3(rst)
  Delay56/1 -> pipeline194/1(d)
  pipeline181/1(q) -> simple_bram_vacc27/1(new_acc)
  pipeline174/1(q) -> simple_bram_vacc26/1(new_acc)
  pipeline171/1(q) -> simple_bram_vacc29/1(new_acc)
  pipeline186/1(q) -> simple_bram_vacc28/1(new_acc)
  pipeline152/1(q) -> simple_bram_vacc28/2(din)
  pipeline169/1(q) -> simple_bram_vacc29/2(din)
  pipeline172/1(q) -> simple_bram_vacc26/2(din)
  pipeline180/1(q) -> simple_bram_vacc27/2(din)
  pipeline182/1(q) -> Counter11/1
  simple_bram_vacc28/2(valid) -> Counter11/2, pipeline187/1(d)
  simple_bram_vacc28/1(dout) -> Reinterpret26/1
  simple_bram_vacc29/1(dout) -> Reinterpret27/1
  simple_bram_vacc26/1(dout) -> Reinterpret28/1
  simple_bram_vacc27/1(dout) -> Reinterpret29/1
  Reinterpret26/1 -> pipeline185/1(d)
  Reinterpret27/1 -> pipeline188/1(d)
  Reinterpret28/1 -> pipeline189/1(d)
  Reinterpret29/1 -> pipeline190/1(d)
  Counter11/1 -> Relational18/2, Relational19/2
  Constant64/1 -> Mux29/2
  Constant43/1 -> Mux28/2
  Constant44/1 -> Mux30/2
  Constant45/1 -> Mux31/2
  simple_bram_vacc27/2(valid) -> Terminator31/1
  pipeline187/1(q) -> Mux31/1, Mux30/1, Mux28/1, Parallel_Dedispersor_v5/1(Valid), pipeline198/1(d), Logical12/1
  pipeline198/1(q) -> pipeline196/1(d)
  Delay31/1 -> pipeline191/1(d)
  Delay40/1 -> pipeline192/1(d)
  Delay41/1 -> pipeline193/1(d)
  acc_cntrl5/1(new_acc) -> pipeline363/1(d)
  pipeline194/1(q) -> pipeline359/1(d)
  pipeline191/1(q) -> pipeline360/1(d)
  pipeline192/1(q) -> pipeline361/1(d)
  pipeline193/1(q) -> pipeline362/1(d)
  pipeline185/1(q) -> Mux29/3
  pipeline188/1(q) -> Mux28/3
  pipeline189/1(q) -> Mux30/3
  pipeline190/1(q) -> Mux31/3
  Mux29/1 -> Parallel_Dedispersor_v5/2(Data1)
  Mux28/1 -> Parallel_Dedispersor_v5/3(Data2)
  Mux30/1 -> Parallel_Dedispersor_v5/4(Data3)
  Mux31/1 -> Parallel_Dedispersor_v5/5(Data4)
  Parallel_Dedispersor_v5/1(Out1) -> pipeline199/1(d)
  Parallel_Dedispersor_v5/2(Out2) -> pipeline200/1(d)
  Parallel_Dedispersor_v5/3(Out3) -> pipeline201/1(d)
  Parallel_Dedispersor_v5/4(Out4) -> pipeline202/1(d)
  pipeline141/1(q) -> Logical12/3
  pipeline124/1(q) -> Logical12/2
  Logical12/1 -> Mux29/1
  Relational18/1 -> pipeline124/1(d)
  Relational19/1 -> pipeline141/1(d)
  Constant48/1 -> Relational18/1
  Constant65/1 -> Relational19/1
  simple_bram_vacc29/2(valid) -> Terminator30/1
  simple_bram_vacc26/2(valid) -> Terminator29/1
  Delay43/1 -> acc_cntrl6/2(sync)
  [acc_len7] -> acc_cntrl6/1(acc_len)
  [cnt_rst] -> acc_cntrl6/3(rst)
  Delay44/1 -> pipeline234/1(d)
  pipeline215/1(q) -> simple_bram_vacc19/1(new_acc)
  pipeline213/1(q) -> simple_bram_vacc18/1(new_acc)
  pipeline211/1(q) -> simple_bram_vacc31/1(new_acc)
  pipeline218/1(q) -> simple_bram_vacc30/1(new_acc)
  pipeline208/1(q) -> simple_bram_vacc30/2(din)
  pipeline210/1(q) -> simple_bram_vacc31/2(din)
  pipeline212/1(q) -> simple_bram_vacc18/2(din)
  pipeline214/1(q) -> simple_bram_vacc19/2(din)
  pipeline216/1(q) -> Counter14/1
  simple_bram_vacc30/2(valid) -> Counter14/2, pipeline219/1(d)
  simple_bram_vacc30/1(dout) -> Reinterpret30/1
  simple_bram_vacc31/1(dout) -> Reinterpret31/1
  simple_bram_vacc18/1(dout) -> Reinterpret18/1
  simple_bram_vacc19/1(dout) -> Reinterpret19/1
  Reinterpret30/1 -> pipeline217/1(d)
  Reinterpret31/1 -> pipeline220/1(d)
  Reinterpret18/1 -> pipeline222/1(d)
  Reinterpret19/1 -> pipeline225/1(d)
  Counter14/1 -> Relational21/2, Relational22/2
  Constant49/1 -> Mux18/2
  Constant56/1 -> Mux32/2
  Constant57/1 -> Mux19/2
  Constant58/1 -> Mux20/2
  simple_bram_vacc19/2(valid) -> Terminator17/1
  pipeline219/1(q) -> Mux20/1, Mux19/1, Mux32/1, Parallel_Dedispersor_v6/1(Valid), pipeline151/1(d), Logical14/1
  pipeline151/1(q) -> pipeline239/1(d)
  Delay47/1 -> pipeline227/1(d)
  Delay48/1 -> pipeline232/1(d)
  Delay49/1 -> pipeline233/1(d)
  acc_cntrl6/1(new_acc) -> pipeline368/1(d)
  pipeline234/1(q) -> pipeline364/1(d)
  pipeline227/1(q) -> pipeline365/1(d)
  pipeline232/1(q) -> pipeline366/1(d)
  pipeline233/1(q) -> pipeline367/1(d)
  pipeline217/1(q) -> Mux18/3
  pipeline220/1(q) -> Mux32/3
  pipeline222/1(q) -> Mux19/3
  pipeline225/1(q) -> Mux20/3
  Mux18/1 -> Parallel_Dedispersor_v6/2(Data1)
  Mux32/1 -> Parallel_Dedispersor_v6/3(Data2)
  Mux19/1 -> Parallel_Dedispersor_v6/4(Data3)
  Mux20/1 -> Parallel_Dedispersor_v6/5(Data4)
  Parallel_Dedispersor_v6/1(Out1) -> pipeline153/1(d)
  Parallel_Dedispersor_v6/2(Out2) -> pipeline154/1(d)
  Parallel_Dedispersor_v6/3(Out3) -> pipeline155/1(d)
  Parallel_Dedispersor_v6/4(Out4) -> pipeline156/1(d)
  pipeline205/1(q) -> Logical14/3
  pipeline204/1(q) -> Logical14/2
  Logical14/1 -> Mux18/1
  Relational21/1 -> pipeline204/1(d)
  Relational22/1 -> pipeline205/1(d)
  Constant47/1 -> Relational21/1
  Constant50/1 -> Relational22/1
  simple_bram_vacc31/2(valid) -> Terminator34/1
  simple_bram_vacc18/2(valid) -> Terminator33/1
  Delay50/1 -> acc_cntrl7/2(sync)
  [acc_len8] -> acc_cntrl7/1(acc_len)
  [cnt_rst] -> acc_cntrl7/3(rst)
  Delay51/1 -> pipeline142/1(d)
  pipeline237/1(q) -> simple_bram_vacc21/1(new_acc)
  pipeline226/1(q) -> simple_bram_vacc20/1(new_acc)
  pipeline223/1(q) -> simple_bram_vacc23/1(new_acc)
  pipeline125/1(q) -> simple_bram_vacc22/1(new_acc)
  pipeline207/1(q) -> simple_bram_vacc22/2(din)
  pipeline221/1(q) -> simple_bram_vacc23/2(din)
  pipeline224/1(q) -> simple_bram_vacc20/2(din)
  pipeline236/1(q) -> simple_bram_vacc21/2(din)
  pipeline238/1(q) -> Counter15/1
  simple_bram_vacc22/2(valid) -> pipeline126/1(d), Counter15/2
  simple_bram_vacc22/1(dout) -> Reinterpret20/1
  simple_bram_vacc23/1(dout) -> Reinterpret21/1
  simple_bram_vacc20/1(dout) -> Reinterpret22/1
  simple_bram_vacc21/1(dout) -> Reinterpret23/1
  Reinterpret20/1 -> pipeline241/1(d)
  Reinterpret21/1 -> pipeline127/1(d)
  Reinterpret22/1 -> pipeline128/1(d)
  Reinterpret23/1 -> pipeline129/1(d)
  Counter15/1 -> Relational15/2, Relational14/2
  Constant59/1 -> Mux22/2
  Constant52/1 -> Mux21/2
  Constant53/1 -> Mux23/2
  Constant54/1 -> Mux24/2
  simple_bram_vacc21/2(valid) -> Terminator24/1
  pipeline126/1(q) -> Mux24/1, Mux23/1, Mux21/1, Parallel_Dedispersor_v7/1(Valid), pipeline146/1(d), Logical16/1
  pipeline146/1(q) -> pipeline144/1(d)
  Delay42/1 -> pipeline130/1(d)
  Delay45/1 -> pipeline131/1(d)
  Delay46/1 -> pipeline132/1(d)
  acc_cntrl7/1(new_acc) -> pipeline373/1(d)
  pipeline142/1(q) -> pipeline369/1(d)
  pipeline130/1(q) -> pipeline370/1(d)
  pipeline131/1(q) -> pipeline371/1(d)
  pipeline132/1(q) -> pipeline372/1(d)
  pipeline241/1(q) -> Mux22/3
  pipeline127/1(q) -> Mux21/3
  pipeline128/1(q) -> Mux23/3
  pipeline129/1(q) -> Mux24/3
  Mux22/1 -> Parallel_Dedispersor_v7/2(Data1)
  Mux21/1 -> Parallel_Dedispersor_v7/3(Data2)
  Mux23/1 -> Parallel_Dedispersor_v7/4(Data3)
  Mux24/1 -> Parallel_Dedispersor_v7/5(Data4)
  Parallel_Dedispersor_v7/1(Out1) -> pipeline147/1(d)
  Parallel_Dedispersor_v7/2(Out2) -> pipeline148/1(d)
  Parallel_Dedispersor_v7/3(Out3) -> pipeline149/1(d)
  Parallel_Dedispersor_v7/4(Out4) -> pipeline150/1(d)
  pipeline206/1(q) -> Logical16/3
  pipeline203/1(q) -> Logical16/2
  Logical16/1 -> Mux22/1
  Relational14/1 -> pipeline203/1(d)
  Relational15/1 -> pipeline206/1(d)
  Constant55/1 -> Relational14/1
  Constant60/1 -> Relational15/1
  simple_bram_vacc23/2(valid) -> Terminator23/1
  simple_bram_vacc20/2(valid) -> Terminator20/1
  Delay58/1 -> acc_cntrl8/2(sync)
  [acc_len9] -> acc_cntrl8/1(acc_len)
  [cnt_rst] -> acc_cntrl8/3(rst)
  Delay59/1 -> pipeline290/1(d)
  pipeline275/1(q) -> simple_bram_vacc33/1(new_acc)
  pipeline273/1(q) -> simple_bram_vacc32/1(new_acc)
  pipeline271/1(q) -> simple_bram_vacc39/1(new_acc)
  pipeline278/1(q) -> simple_bram_vacc38/1(new_acc)
  pipeline269/1(q) -> simple_bram_vacc38/2(din)
  pipeline270/1(q) -> simple_bram_vacc39/2(din)
  pipeline272/1(q) -> simple_bram_vacc32/2(din)
  pipeline274/1(q) -> simple_bram_vacc33/2(din)
  pipeline276/1(q) -> Counter18/1
  simple_bram_vacc38/2(valid) -> pipeline279/1(d), Counter18/2
  simple_bram_vacc38/1(dout) -> Reinterpret38/1
  simple_bram_vacc39/1(dout) -> Reinterpret39/1
  simple_bram_vacc32/1(dout) -> Reinterpret32/1
  simple_bram_vacc33/1(dout) -> Reinterpret33/1
  Reinterpret38/1 -> pipeline277/1(d)
  Reinterpret39/1 -> pipeline280/1(d)
  Reinterpret32/1 -> pipeline282/1(d)
  Reinterpret33/1 -> pipeline285/1(d)
  Counter18/1 -> Relational28/2, Relational27/2
  Constant68/1 -> Mux33/2
  Constant75/1 -> Mux40/2
  Constant76/1 -> Mux34/2
  Constant77/1 -> Mux35/2
  simple_bram_vacc33/2(valid) -> Terminator35/1
  pipeline279/1(q) -> Mux35/1, Mux34/1, Mux40/1, Parallel_Dedispersor_v8/1(Valid), pipeline259/1(d), Logical18/1
  pipeline259/1(q) -> pipeline295/1(d)
  Delay62/1 -> pipeline287/1(d)
  Delay63/1 -> pipeline288/1(d)
  Delay64/1 -> pipeline289/1(d)
  acc_cntrl8/1(new_acc) -> pipeline378/1(d)
  pipeline290/1(q) -> pipeline374/1(d)
  pipeline287/1(q) -> pipeline375/1(d)
  pipeline288/1(q) -> pipeline376/1(d)
  pipeline289/1(q) -> pipeline377/1(d)
  pipeline277/1(q) -> Mux33/3
  pipeline280/1(q) -> Mux40/3
  pipeline282/1(q) -> Mux34/3
  pipeline285/1(q) -> Mux35/3
  Mux33/1 -> Parallel_Dedispersor_v8/2(Data1)
  Mux40/1 -> Parallel_Dedispersor_v8/3(Data2)
  Mux34/1 -> Parallel_Dedispersor_v8/4(Data3)
  Mux35/1 -> Parallel_Dedispersor_v8/5(Data4)
  Parallel_Dedispersor_v8/1(Out1) -> pipeline260/1(d)
  Parallel_Dedispersor_v8/2(Out2) -> pipeline261/1(d)
  Parallel_Dedispersor_v8/3(Out3) -> pipeline262/1(d)
  Parallel_Dedispersor_v8/4(Out4) -> pipeline263/1(d)
  pipeline266/1(q) -> Logical18/3
  pipeline265/1(q) -> Logical18/2
  Logical18/1 -> Mux33/1
  Relational27/1 -> pipeline265/1(d)
  Relational28/1 -> pipeline266/1(d)
  Constant67/1 -> Relational27/1
  Constant69/1 -> Relational28/1
  simple_bram_vacc39/2(valid) -> Terminator42/1
  simple_bram_vacc32/2(valid) -> Terminator41/1
  Delay65/1 -> acc_cntrl9/2(sync)
  [acc_len10] -> acc_cntrl9/1(acc_len)
  [cnt_rst] -> acc_cntrl9/3(rst)
  Delay66/1 -> pipeline250/1(d)
  pipeline293/1(q) -> simple_bram_vacc35/1(new_acc)
  pipeline286/1(q) -> simple_bram_vacc34/1(new_acc)
  pipeline283/1(q) -> simple_bram_vacc37/1(new_acc)
  pipeline242/1(q) -> simple_bram_vacc36/1(new_acc)
  pipeline268/1(q) -> simple_bram_vacc36/2(din)
  pipeline281/1(q) -> simple_bram_vacc37/2(din)
  pipeline284/1(q) -> simple_bram_vacc34/2(din)
  pipeline292/1(q) -> simple_bram_vacc35/2(din)
  pipeline294/1(q) -> Counter19/1
  simple_bram_vacc36/2(valid) -> Counter19/2, pipeline243/1(d)
  simple_bram_vacc36/1(dout) -> Reinterpret34/1
  simple_bram_vacc37/1(dout) -> Reinterpret35/1
  simple_bram_vacc34/1(dout) -> Reinterpret36/1
  simple_bram_vacc35/1(dout) -> Reinterpret37/1
  Reinterpret34/1 -> pipeline297/1(d)
  Reinterpret35/1 -> pipeline244/1(d)
  Reinterpret36/1 -> pipeline245/1(d)
  Reinterpret37/1 -> pipeline246/1(d)
  Counter19/1 -> Relational24/2, Relational25/2
  Constant78/1 -> Mux37/2
  Constant71/1 -> Mux36/2
  Constant72/1 -> Mux38/2
  Constant73/1 -> Mux39/2
  simple_bram_vacc35/2(valid) -> Terminator39/1
  pipeline243/1(q) -> Mux39/1, Mux38/1, Mux36/1, Parallel_Dedispersor_v9/1(Valid), pipeline254/1(d), Logical20/1
  pipeline254/1(q) -> pipeline252/1(d)
  Delay57/1 -> pipeline247/1(d)
  Delay60/1 -> pipeline248/1(d)
  Delay61/1 -> pipeline249/1(d)
  acc_cntrl9/1(new_acc) -> pipeline383/1(d)
  pipeline250/1(q) -> pipeline379/1(d)
  pipeline247/1(q) -> pipeline380/1(d)
  pipeline248/1(q) -> pipeline381/1(d)
  pipeline249/1(q) -> pipeline382/1(d)
  pipeline297/1(q) -> Mux37/3
  pipeline244/1(q) -> Mux36/3
  pipeline245/1(q) -> Mux38/3
  pipeline246/1(q) -> Mux39/3
  Mux37/1 -> Parallel_Dedispersor_v9/2(Data1)
  Mux36/1 -> Parallel_Dedispersor_v9/3(Data2)
  Mux38/1 -> Parallel_Dedispersor_v9/4(Data3)
  Mux39/1 -> Parallel_Dedispersor_v9/5(Data4)
  Parallel_Dedispersor_v9/1(Out1) -> pipeline255/1(d)
  Parallel_Dedispersor_v9/2(Out2) -> pipeline256/1(d)
  Parallel_Dedispersor_v9/3(Out3) -> pipeline257/1(d)
  Parallel_Dedispersor_v9/4(Out4) -> pipeline258/1(d)
  pipeline267/1(q) -> Logical20/3
  pipeline264/1(q) -> Logical20/2
  Logical20/1 -> Mux37/1
  Relational24/1 -> pipeline264/1(d)
  Relational25/1 -> pipeline267/1(d)
  Constant74/1 -> Relational24/1
  Constant79/1 -> Relational25/1
  simple_bram_vacc37/2(valid) -> Terminator38/1
  simple_bram_vacc34/2(valid) -> Terminator37/1
  power1/1 -> Delay67/1
  power3/1 -> Delay70/1
  Constant82/1 -> gain/1(sim_1)
  gain/1(in_reg) -> pipeline302/1(d)
  pipeline302/1(q) -> [gain]
  [gain] -> Mult/2
  [gain] -> Mult1/2
  [gain] -> Mult2/2
  [gain] -> Mult3/2
  Delay71/1 -> pipeline347/1(d), Delay75/1
  Delay69/1 -> pipeline345/1(d), Delay73/1
  Delay76/1 -> acc_cntrl11/2(sync)
  [acc_len] -> acc_cntrl11/1(acc_len)
  [cnt_rst] -> acc_cntrl11/3(rst)
  Delay72/1 -> pipeline304/1(d)
  pipeline315/1(q) -> simple_bram_vacc46/1(new_acc)
  pipeline311/1(q) -> simple_bram_vacc46/2(din)
  pipeline314/1(q) -> Counter22/1
  acc_cntrl11/1(new_acc) -> pipeline398/1(d)
  pipeline304/1(q) -> pipeline394/1(d)
  simple_bram_vacc46/1(dout) -> Reinterpret40/1
  spec1_0/1(data_out) -> Terminator46/1
  simple_bram_vacc46/2(valid) -> spec1_0/3(we), Counter22/2
  pipeline305/1(q) -> simple_bram_vacc43/1(new_acc)
  pipeline303/1(q) -> simple_bram_vacc43/2(din)
  simple_bram_vacc43/1(dout) -> Reinterpret41/1
  spec1_1/1(data_out) -> Terminator43/1
  simple_bram_vacc43/2(valid) -> spec1_1/3(we)
  pipeline309/1(q) -> simple_bram_vacc45/1(new_acc)
  pipeline308/1(q) -> simple_bram_vacc45/2(din)
  simple_bram_vacc45/1(dout) -> Reinterpret42/1
  spec1_2/1(data_out) -> Terminator45/1
  simple_bram_vacc45/2(valid) -> spec1_2/3(we)
  pipeline307/1(q) -> simple_bram_vacc44/1(new_acc)
  pipeline306/1(q) -> simple_bram_vacc44/2(din)
  simple_bram_vacc44/1(dout) -> Reinterpret43/1
  spec1_3/1(data_out) -> Terminator44/1
  simple_bram_vacc44/2(valid) -> spec1_3/3(we)
  Counter22/1 -> spec1_0/1(addr), spec1_1/1(addr), spec1_2/1(addr), spec1_3/1(addr)
  Delay73/1 -> pipeline310/1(d)
  pipeline310/1(q) -> pipeline395/1(d)
  Delay74/1 -> pipeline312/1(d)
  pipeline312/1(q) -> pipeline396/1(d)
  Delay75/1 -> pipeline313/1(d)
  pipeline313/1(q) -> pipeline397/1(d)
  Delay68/1 -> pipeline351/1(d), Delay76/1
  Delay67/1 -> pipeline348/1(d), Delay72/1
  Delay70/1 -> pipeline346/1(d), Delay74/1
  Delay80/1 -> acc_cntrl12/2(sync)
  [acc_len0] -> acc_cntrl12/1(acc_len)
  [cnt_rst] -> acc_cntrl12/3(rst)
  Delay81/1 -> pipeline324/1(d)
  pipeline341/1(q) -> simple_bram_vacc48/1(new_acc)
  pipeline339/1(q) -> simple_bram_vacc47/1(new_acc)
  pipeline337/1(q) -> simple_bram_vacc50/1(new_acc)
  pipeline316/1(q) -> simple_bram_vacc49/1(new_acc)
  pipeline335/1(q) -> simple_bram_vacc49/2(din)
  pipeline336/1(q) -> simple_bram_vacc50/2(din)
  pipeline338/1(q) -> simple_bram_vacc47/2(din)
  pipeline340/1(q) -> simple_bram_vacc48/2(din)
  pipeline342/1(q) -> Counter24/1
  simple_bram_vacc49/2(valid) -> pipeline317/1(d), Counter24/2
  simple_bram_vacc49/1(dout) -> Reinterpret44/1
  simple_bram_vacc50/1(dout) -> Reinterpret45/1
  simple_bram_vacc47/1(dout) -> Reinterpret46/1
  simple_bram_vacc48/1(dout) -> Reinterpret47/1
  Reinterpret44/1 -> pipeline343/1(d)
  Reinterpret45/1 -> pipeline318/1(d)
  Reinterpret46/1 -> pipeline319/1(d)
  Reinterpret47/1 -> pipeline320/1(d)
  Counter24/1 -> Relational31/2, Relational30/2
  Constant91/1 -> Mux42/2
  Constant84/1 -> Mux41/2
  Constant85/1 -> Mux43/2
  Constant86/1 -> Mux44/2
  pipeline326/1(q) -> adder_tree10/1(sync)
  edge_detect10/1 -> Logical21/1, Accumulator10/2
  adder_tree10/1(sync_out) -> Accumulator10/3, edge_detect10/1
  adder_tree10/2(dout) -> Accumulator10/1
  Register10/1 -> [frb_detector_0]
  [cnt_rst] -> Register10/2
  Relational32/1 -> Register10/1, Register10/3
  simple_bram_vacc48/2(valid) -> Terminator49/1
  pipeline317/1(q) -> Mux44/1, Mux43/1, Mux41/1, pipeline328/1(d), Logical22/1
  pipeline328/1(q) -> pipeline326/1(d)
  Accumulator10/1 -> Relational32/2, ACC0/2(data_in)
  Counter23/1 -> ACC0/1(addr)
  ACC0/1(data_out) -> Terminator50/1
  Logical21/1 -> Counter23/1
  Delay77/1 -> pipeline321/1(d)
  Delay78/1 -> pipeline322/1(d)
  Delay79/1 -> pipeline323/1(d)
  acc_cntrl12/1(new_acc) -> pipeline388/1(d)
  pipeline324/1(q) -> pipeline384/1(d)
  pipeline321/1(q) -> pipeline385/1(d)
  pipeline322/1(q) -> pipeline386/1(d)
  pipeline323/1(q) -> pipeline387/1(d)
  pipeline343/1(q) -> Mux42/3
  pipeline318/1(q) -> Mux41/3
  pipeline319/1(q) -> Mux43/3
  pipeline320/1(q) -> Mux44/3
  Mux42/1 -> pipeline329/1(d)
  Mux41/1 -> pipeline330/1(d)
  Mux43/1 -> pipeline331/1(d)
  Mux44/1 -> pipeline332/1(d)
  pipeline329/1(q) -> pipeline37/1(d)
  pipeline330/1(q) -> pipeline42/1(d)
  pipeline331/1(q) -> pipeline53/1(d)
  pipeline332/1(q) -> pipeline55/1(d)
  pipeline334/1(q) -> Logical22/3
  pipeline333/1(q) -> Logical22/2
  Logical22/1 -> Mux42/1
  Relational30/1 -> pipeline333/1(d)
  Relational31/1 -> pipeline334/1(d)
  Constant90/1 -> Relational30/1
  Constant92/1 -> Relational31/1
  Constant83/1 -> Logical21/2
  theta0/1(in_reg) -> Convert11/1
  Convert11/1 -> Relational32/1
  simple_bram_vacc50/2(valid) -> Terminator48/1
  simple_bram_vacc47/2(valid) -> Terminator47/1
  Constant93/1 -> acc_len0/1(sim_1)
  acc_len0/1(in_reg) -> pipeline344/1(d)
  pipeline344/1(q) -> [acc_len0]
  Convert12/1 -> spec0_0/2(data_in)
  Convert13/1 -> spec0_1/2(data_in)
  Convert14/1 -> spec0_2/2(data_in)
  Convert15/1 -> spec0_3/2(data_in)
  Reinterpret40/1 -> spec1_0/2(data_in)
  Reinterpret41/1 -> spec1_1/2(data_in)
  Reinterpret42/1 -> spec1_2/2(data_in)
  Reinterpret43/1 -> spec1_3/2(data_in)
  pipeline345/1(q) -> Mult1/1
  pipeline348/1(q) -> Mult/1
  pipeline346/1(q) -> Mult2/1
  pipeline347/1(q) -> Mult3/1
  pipeline351/1(q) -> pipeline350/1(d)
  pipeline41/1(q) -> adder_tree/1(sync)
  Constant10/1 -> ACC1/3(we)
  edge_detect1/1 -> Logical3/1, Accumulator1/2
  adder_tree1/1(sync_out) -> edge_detect1/1, Accumulator1/3
  adder_tree1/2(dout) -> Accumulator1/1
  Register1/1 -> [frb_detector_2]
  [cnt_rst] -> Register1/2
  Relational3/1 -> Register1/1, Register1/3
  Accumulator1/1 -> ACC2/2(data_in), Relational3/2
  Counter2/1 -> ACC2/1(addr)
  ACC2/1(data_out) -> Terminator7/1
  Logical3/1 -> Counter2/1
  pipeline57/1(q) -> adder_tree1/2(din1)
  pipeline58/1(q) -> adder_tree1/3(din2)
  pipeline59/1(q) -> adder_tree1/4(din3)
  pipeline60/1(q) -> adder_tree1/5(din4)
  Constant22/1 -> Logical3/2
  theta2/1(in_reg) -> Convert2/1
  Convert2/1 -> Relational3/1
  pipeline54/1(q) -> adder_tree1/1(sync)
  Constant18/1 -> ACC2/3(we)
  edge_detect2/1 -> Logical5/1, Accumulator2/2
  adder_tree2/1(sync_out) -> edge_detect2/1, Accumulator2/3
  adder_tree2/2(dout) -> Accumulator2/1
  Register2/1 -> [frb_detector_3]
  [cnt_rst] -> Register2/2
  Relational6/1 -> Register2/1, Register2/3
  Accumulator2/1 -> ACC3/2(data_in), Relational6/2
  Counter4/1 -> ACC3/1(addr)
  ACC3/1(data_out) -> Terminator11/1
  Logical5/1 -> Counter4/1
  pipeline120/1(q) -> adder_tree2/2(din1)
  pipeline121/1(q) -> adder_tree2/3(din2)
  pipeline122/1(q) -> adder_tree2/4(din3)
  pipeline123/1(q) -> adder_tree2/5(din4)
  Constant42/1 -> Logical5/2
  theta3/1(in_reg) -> Convert3/1
  Convert3/1 -> Relational6/1
  pipeline97/1(q) -> adder_tree2/1(sync)
  Constant38/1 -> ACC3/3(we)
  edge_detect3/1 -> Accumulator3/2, Logical7/1
  adder_tree3/1(sync_out) -> Accumulator3/3, edge_detect3/1
  adder_tree3/2(dout) -> Accumulator3/1
  Register3/1 -> [frb_detector_4]
  [cnt_rst] -> Register3/2
  Relational9/1 -> Register3/3, Register3/1
  Accumulator3/1 -> Relational9/2, ACC4/2(data_in)
  Counter5/1 -> ACC4/1(addr)
  ACC4/1(data_out) -> Terminator15/1
  Logical7/1 -> Counter5/1
  pipeline115/1(q) -> adder_tree3/2(din1)
  pipeline116/1(q) -> adder_tree3/3(din2)
  pipeline117/1(q) -> adder_tree3/4(din3)
  pipeline118/1(q) -> adder_tree3/5(din4)
  Constant51/1 -> Logical7/2
  theta4/1(in_reg) -> Convert4/1
  Convert4/1 -> Relational9/1
  pipeline112/1(q) -> adder_tree3/1(sync)
  Constant46/1 -> ACC4/3(we)
  edge_detect4/1 -> Logical9/1, Accumulator4/2
  adder_tree4/1(sync_out) -> edge_detect4/1, Accumulator4/3
  adder_tree4/2(dout) -> Accumulator4/1
  Register4/1 -> [frb_detector_5]
  [cnt_rst] -> Register4/2
  Relational12/1 -> Register4/1, Register4/3
  Accumulator4/1 -> ACC5/2(data_in), Relational12/2
  Counter8/1 -> ACC5/1(addr)
  ACC5/1(data_out) -> Terminator28/1
  Logical9/1 -> Counter8/1
  pipeline228/1(q) -> adder_tree4/2(din1)
  pipeline229/1(q) -> adder_tree4/3(din2)
  pipeline230/1(q) -> adder_tree4/4(din3)
  pipeline231/1(q) -> adder_tree4/5(din4)
  Constant70/1 -> Logical9/2
  theta5/1(in_reg) -> Convert5/1
  Convert5/1 -> Relational12/1
  pipeline183/1(q) -> adder_tree4/1(sync)
  Constant66/1 -> ACC5/3(we)
  edge_detect5/1 -> Accumulator5/2, Logical11/1
  adder_tree5/1(sync_out) -> Accumulator5/3, edge_detect5/1
  adder_tree5/2(dout) -> Accumulator5/1
  Register5/1 -> [frb_detector_6]
  [cnt_rst] -> Register5/2
  Relational17/1 -> Register5/3, Register5/1
  Accumulator5/1 -> Relational17/2, ACC6/2(data_in)
  Counter9/1 -> ACC6/1(addr)
  ACC6/1(data_out) -> Terminator32/1
  Logical11/1 -> Counter9/1
  pipeline199/1(q) -> adder_tree5/2(din1)
  pipeline200/1(q) -> adder_tree5/3(din2)
  pipeline201/1(q) -> adder_tree5/4(din3)
  pipeline202/1(q) -> adder_tree5/5(din4)
  Constant95/1 -> Logical11/2
  theta6/1(in_reg) -> Convert6/1
  Convert6/1 -> Relational17/1
  pipeline196/1(q) -> adder_tree5/1(sync)
  Constant94/1 -> ACC6/3(we)
  edge_detect6/1 -> Accumulator6/2, Logical13/1
  adder_tree6/1(sync_out) -> Accumulator6/3, edge_detect6/1
  adder_tree6/2(dout) -> Accumulator6/1
  Register6/1 -> [frb_detector_7]
  [cnt_rst] -> Register6/2
  Relational20/1 -> Register6/3, Register6/1
  Accumulator6/1 -> Relational20/2, ACC7/2(data_in)
  Counter12/1 -> ACC7/1(addr)
  ACC7/1(data_out) -> Terminator19/1
  Logical13/1 -> Counter12/1
  pipeline153/1(q) -> adder_tree6/2(din1)
  pipeline154/1(q) -> adder_tree6/3(din2)
  pipeline155/1(q) -> adder_tree6/4(din3)
  pipeline156/1(q) -> adder_tree6/5(din4)
  Constant97/1 -> Logical13/2
  theta7/1(in_reg) -> Convert7/1
  Convert7/1 -> Relational20/1
  pipeline239/1(q) -> adder_tree6/1(sync)
  Constant96/1 -> ACC7/3(we)
  edge_detect7/1 -> Logical15/1, Accumulator7/2
  adder_tree7/1(sync_out) -> edge_detect7/1, Accumulator7/3
  adder_tree7/2(dout) -> Accumulator7/1
  Register7/1 -> [frb_detector_8]
  [cnt_rst] -> Register7/2
  Relational23/1 -> Register7/1, Register7/3
  Accumulator7/1 -> ACC8/2(data_in), Relational23/2
  Counter13/1 -> ACC8/1(addr)
  ACC8/1(data_out) -> Terminator25/1
  Logical15/1 -> Counter13/1
  pipeline147/1(q) -> adder_tree7/2(din1)
  pipeline148/1(q) -> adder_tree7/3(din2)
  pipeline149/1(q) -> adder_tree7/4(din3)
  pipeline150/1(q) -> adder_tree7/5(din4)
  Constant99/1 -> Logical15/2
  theta8/1(in_reg) -> Convert8/1
  Convert8/1 -> Relational23/1
  pipeline144/1(q) -> adder_tree7/1(sync)
  Constant98/1 -> ACC8/3(we)
  edge_detect8/1 -> Logical17/1, Accumulator8/2
  adder_tree8/1(sync_out) -> edge_detect8/1, Accumulator8/3
  adder_tree8/2(dout) -> Accumulator8/1
  Register8/1 -> [frb_detector_9]
  [cnt_rst] -> Register8/2
  Relational26/1 -> Register8/1, Register8/3
  Accumulator8/1 -> ACC9/2(data_in), Relational26/2
  Counter16/1 -> ACC9/1(addr)
  ACC9/1(data_out) -> Terminator36/1
  Logical17/1 -> Counter16/1
  pipeline260/1(q) -> adder_tree8/2(din1)
  pipeline261/1(q) -> adder_tree8/3(din2)
  pipeline262/1(q) -> adder_tree8/4(din3)
  pipeline263/1(q) -> adder_tree8/5(din4)
  Constant101/1 -> Logical17/2
  theta9/1(in_reg) -> Convert9/1
  Convert9/1 -> Relational26/1
  pipeline295/1(q) -> adder_tree8/1(sync)
  Constant100/1 -> ACC9/3(we)
  edge_detect9/1 -> Accumulator9/2, Logical19/1
  adder_tree9/1(sync_out) -> Accumulator9/3, edge_detect9/1
  adder_tree9/2(dout) -> Accumulator9/1
  Register9/1 -> [frb_detector_10]
  [cnt_rst] -> Register9/2
  Relational29/1 -> Register9/3, Register9/1
  Accumulator9/1 -> Relational29/2, ACC10/2(data_in)
  Counter17/1 -> ACC10/1(addr)
  ACC10/1(data_out) -> Terminator40/1
  Logical19/1 -> Counter17/1
  pipeline255/1(q) -> adder_tree9/2(din1)
  pipeline256/1(q) -> adder_tree9/3(din2)
  pipeline257/1(q) -> adder_tree9/4(din3)
  pipeline258/1(q) -> adder_tree9/5(din4)
  Constant103/1 -> Logical19/2
  theta10/1(in_reg) -> Convert10/1
  Convert10/1 -> Relational29/1
  pipeline252/1(q) -> adder_tree9/1(sync)
  Constant102/1 -> ACC10/3(we)
  pipeline37/1(q) -> adder_tree10/2(din1)
  pipeline42/1(q) -> adder_tree10/3(din2)
  pipeline53/1(q) -> adder_tree10/4(din3)
  pipeline55/1(q) -> adder_tree10/5(din4)
  Constant104/1 -> ACC0/3(we)
  pipeline93/1(q) -> pipeline40/1(d), pipeline44/1(d), pipeline27/1(d), pipeline30/1(d), pipeline39/1(d)
  pipeline98/1(q) -> pipeline22/1(d), pipeline19/1(d), pipeline17/1(d), pipeline15/1(d), pipeline20/1(d)
  pipeline111/1(q) -> pipeline13/1(d)
  pipeline113/1(q) -> pipeline14/1(d)
  pipeline143/1(q) -> pipeline16/1(d)
  pipeline145/1(q) -> pipeline18/1(d)
  pipeline179/1(q) -> pipeline12/1(d)
  pipeline184/1(q) -> pipeline25/1(d)
  pipeline195/1(q) -> pipeline28/1(d)
  pipeline197/1(q) -> pipeline38/1(d)
  pipeline240/1(q) -> pipeline68/1(d)
  pipeline291/1(q) -> pipeline74/1(d), pipeline73/1(d), pipeline71/1(d), pipeline69/1(d), pipeline76/1(d)
  pipeline251/1(q) -> pipeline70/1(d)
  pipeline253/1(q) -> pipeline72/1(d)
  pipeline235/1(q) -> pipeline66/1(d)
  pipeline325/1(q) -> pipeline79/1(d)
  pipeline353/1(q) -> pipeline100/1(d), pipeline81/1(d), pipeline95/1(d), pipeline84/1(d), pipeline96/1(d)
  pipeline327/1(q) -> pipeline82/1(d)
  pipeline296/1(q) -> pipeline65/1(d)
  pipeline352/1(q) -> pipeline94/1(d)
  pipeline355/1(q) -> pipeline158/1(d)
  pipeline357/1(q) -> pipeline162/1(d)
  pipeline356/1(q) -> pipeline160/1(d)
  pipeline354/1(q) -> pipeline157/1(d)
  pipeline358/1(q) -> pipeline164/1(d), pipeline161/1(d), pipeline163/1(d), pipeline159/1(d), pipeline166/1(d)
  pipeline359/1(q) -> pipeline152/1(d)
  pipeline361/1(q) -> pipeline172/1(d)
  pipeline360/1(q) -> pipeline169/1(d)
  pipeline362/1(q) -> pipeline180/1(d)
  pipeline363/1(q) -> pipeline186/1(d), pipeline171/1(d), pipeline181/1(d), pipeline174/1(d), pipeline182/1(d)
  pipeline368/1(q) -> pipeline218/1(d), pipeline211/1(d), pipeline215/1(d), pipeline213/1(d), pipeline216/1(d)
  pipeline365/1(q) -> pipeline210/1(d)
  pipeline364/1(q) -> pipeline208/1(d)
  pipeline367/1(q) -> pipeline214/1(d)
  pipeline366/1(q) -> pipeline212/1(d)
  pipeline372/1(q) -> pipeline236/1(d)
  pipeline370/1(q) -> pipeline221/1(d)
  pipeline373/1(q) -> pipeline238/1(d), pipeline237/1(d), pipeline226/1(d), pipeline223/1(d), pipeline125/1(d)
  pipeline371/1(q) -> pipeline224/1(d)
  pipeline369/1(q) -> pipeline207/1(d)
  pipeline376/1(q) -> pipeline272/1(d)
  pipeline375/1(q) -> pipeline270/1(d)
  pipeline377/1(q) -> pipeline274/1(d)
  pipeline378/1(q) -> pipeline276/1(d), pipeline275/1(d), pipeline273/1(d), pipeline271/1(d), pipeline278/1(d)
  pipeline374/1(q) -> pipeline269/1(d)
  pipeline382/1(q) -> pipeline292/1(d)
  pipeline381/1(q) -> pipeline284/1(d)
  pipeline379/1(q) -> pipeline268/1(d)
  pipeline380/1(q) -> pipeline281/1(d)
  pipeline383/1(q) -> pipeline293/1(d), pipeline286/1(d), pipeline283/1(d), pipeline242/1(d), pipeline294/1(d)
  pipeline387/1(q) -> pipeline340/1(d)
  pipeline386/1(q) -> pipeline338/1(d)
  pipeline388/1(q) -> pipeline342/1(d), pipeline341/1(d), pipeline339/1(d), pipeline337/1(d), pipeline316/1(d)
  pipeline384/1(q) -> pipeline335/1(d)
  pipeline385/1(q) -> pipeline336/1(d)
  pipeline389/1(q) -> pipeline617/1(d)
  pipeline391/1(q) -> pipeline606/1(d)
  pipeline392/1(q) -> pipeline604/1(d)
  pipeline390/1(q) -> pipeline601/1(d)
  pipeline393/1(q) -> pipeline605/1(d), pipeline607/1(d), pipeline603/1(d), pipeline625/1(d), pipeline624/1(d)
  pipeline397/1(q) -> pipeline306/1(d)
  pipeline394/1(q) -> pipeline311/1(d)
  pipeline396/1(q) -> pipeline308/1(d)
  pipeline395/1(q) -> pipeline303/1(d)
  pipeline398/1(q) -> pipeline314/1(d), pipeline307/1(d), pipeline309/1(d), pipeline305/1(d), pipeline315/1(d)
  [m0d0] -> Delay13/1
  [m0d1] -> Delay8/1
  [m0d2] -> Delay21/1
  [m0d3] -> Delay30/1
  [m0d4] -> Delay39/1
  [m0d5] -> Delay56/1
  [m0d6] -> Delay44/1
  [m0d7] -> Delay51/1
  [m0d8] -> Delay59/1
  [m0d9] -> Delay66/1
  [m0d10] -> Delay81/1
  [m0d11] -> Delay119/1
  Mult/1 -> m0_tree/1(In1)
  pipeline350/1(q) -> sync_tree/1(In1)
  Mult1/1 -> m1_tree/1(In1)
  Mult2/1 -> m2_tree/1(In1)
  Mult3/1 -> m3_tree/1(In1)
  [sd0] -> Delay12/1
  [m1d0] -> Delay33/1
  [m2d0] -> Delay35/1
  [m3d0] -> Delay37/1
  [sd1] -> Delay5/1
  [m1d1] -> Delay10/1
  [m2d1] -> Delay14/1
  [m3d1] -> Delay15/1
  [sd2] -> Delay19/1
  [m1d2] -> Delay26/1
  [m2d2] -> Delay27/1
  [m3d2] -> Delay28/1
  [sd3] -> Delay29/1
  [m1d3] -> Delay18/1
  [m2d3] -> Delay24/1
  [m3d3] -> Delay25/1
  [sd4] -> Delay32/1
  [m1d4] -> Delay52/1
  [m2d4] -> Delay53/1
  [m3d4] -> Delay54/1
  [sd5] -> Delay55/1
  [m1d5] -> Delay31/1
  [m2d5] -> Delay40/1
  [m3d5] -> Delay41/1
  [sd6] -> Delay43/1
  [m1d6] -> Delay47/1
  [m2d6] -> Delay48/1
  [m3d6] -> Delay49/1
  [sd7] -> Delay50/1
  [m1d7] -> Delay42/1
  [m2d7] -> Delay45/1
  [m3d7] -> Delay46/1
  [sd8] -> Delay58/1
  [m1d8] -> Delay62/1
  [m2d8] -> Delay63/1
  [m3d8] -> Delay64/1
  [sd9] -> Delay65/1
  [m1d9] -> Delay57/1
  [m2d9] -> Delay60/1
  [m3d9] -> Delay61/1
  [sd10] -> Delay80/1
  [m1d10] -> Delay77/1
  [m2d10] -> Delay78/1
  [m3d10] -> Delay79/1
  [sd11] -> Delay127/1
  [m1d11] -> Delay120/1
  [m2d11] -> Delay121/1
  [m3d11] -> Delay122/1
  [rst] -> pipeline421/1
  [rst] -> pipeline422/1
  [gbe_data] -> pipeline423/1
  [gbe_valid] -> pipeline424/1
  [gbe_eof] -> pipeline430/1
  Constant105/1 -> one_GbE/8
  [gbe_dest_ip] -> pipeline428/1
  [gbe_dest_port] -> pipeline429/1
  one_GbE/1 -> Terminator59/1
  one_GbE/2 -> Terminator60/1
  one_GbE/3 -> Terminator61/1
  one_GbE/4 -> Terminator53/1
  one_GbE/5 -> Terminator54/1
  one_GbE/6 -> Terminator55/1
  one_GbE/7 -> Terminator56/1
  one_GbE/8 -> Terminator57/1
  one_GbE/9 -> Terminator58/1
  one_GbE/10 -> Terminator51/1
  one_GbE/11 -> Terminator52/1
  Concat/1 -> pipeline406/1
  ring/1(dout) -> pipeline403/1
  ring/2(eof) -> pipeline404/1
  ring/3(val) -> pipeline405/1
  pipeline407/1 -> Concat/1
  pipeline408/1 -> Concat/2
  pipeline409/1 -> Concat/3
  pipeline406/1 -> ring/2(data_in)
  [adc0_a] -> pipeline407/1
  [adc0_c] -> pipeline408/1
  [adc1_a] -> pipeline409/1
  gbe_dest_port/1(in_reg) -> Delay92/1
  gbe_dest_ip/1(in_reg) -> Delay91/1
  control/1(in_reg) -> Slice3/1, Slice2/1, Slice1/1
  Slice1/1 -> Delay86/1
  Slice2/1 -> Delay87/1
  Delay86/1 -> [write]
  Delay87/1 -> [rst]
  pipeline298/1 -> [adc1_a], [adc0_c], [adc0_a]
  conv_bus0/9(q8) -> pipeline298/1
  pipeline299/1 -> pipeline8/1(d), bus_create0/8(in8)
  pipeline300/1 -> pipeline7/1(d), bus_create0/7(in7)
  pipeline301/1 -> pipeline1/1(d), bus_create0/1(in1)
  pipeline349/1 -> pipeline2/1(d), bus_create0/2(in2)
  pipeline399/1 -> pipeline3/1(d), bus_create0/3(in3)
  pipeline400/1 -> pipeline4/1(d), bus_create0/4(in4)
  pipeline401/1 -> pipeline5/1(d), bus_create0/5(in5)
  pipeline402/1 -> pipeline6/1(d), bus_create0/6(in6)
  Slice3/1 -> Delay88/1
  [frb_detector_0] -> pipeline420/1
  [frb_detector_1] -> pipeline419/1
  [frb_detector_2] -> pipeline418/1
  [frb_detector_3] -> pipeline417/1
  [frb_detector_4] -> pipeline416/1
  [frb_detector_5] -> pipeline415/1
  [frb_detector_6] -> pipeline414/1
  [frb_detector_7] -> pipeline413/1
  [frb_detector_8] -> pipeline412/1
  [frb_detector_9] -> pipeline411/1
  [frb_detector_10] -> pipeline410/1
  Concat1/1 -> Convert/1
  Convert/1 -> frb_detector/1(out_reg)
  Logical/1 -> pipeline/1
  Delay88/1 -> [allow_detect]
  [detection] -> Delay93/1
  [write] -> Logical24/2
  Logical23/1 -> Logical24/1
  [allow_detect] -> Inverter/1
  Logical24/1 -> ring/1(write_en)
  Inverter/1 -> Logical23/1
  pipeline403/1 -> [gbe_data]
  pipeline404/1 -> [gbe_eof]
  pipeline405/1 -> [gbe_valid]
  Delay91/1 -> [gbe_dest_ip]
  Delay92/1 -> [gbe_dest_port]
  Delay93/1 -> Logical23/2
  pipeline/1 -> gpio/1, [detection]
  pipeline410/1 -> Logical/1, Concat1/1
  pipeline411/1 -> Logical/2, Concat1/2
  pipeline412/1 -> Logical/3, Concat1/3
  pipeline413/1 -> Logical/4, Concat1/4
  pipeline414/1 -> Logical/5, Concat1/5
  pipeline415/1 -> Logical/6, Concat1/6
  pipeline416/1 -> Logical/7, Concat1/7
  pipeline417/1 -> Logical/8, Concat1/8
  pipeline418/1 -> Logical/9, Concat1/9
  pipeline419/1 -> Logical/10, Concat1/10
  pipeline420/1 -> Logical/11, Concat1/11
  pipeline421/1 -> one_GbE/1
  pipeline422/1 -> one_GbE/2
  pipeline423/1 -> one_GbE/3
  pipeline424/1 -> one_GbE/4
  pipeline428/1 -> one_GbE/5
  pipeline429/1 -> one_GbE/6
  pipeline430/1 -> one_GbE/7
